simulink library "Centralized_I_Lib_Controller"  (R2024b)
(part 7 of 7)

tau = ft_14({dq1,dq2,dq3,dq4,dq5,dq6,t10,t1004,t1005,t1006,t1007,t1009,t101,t1010,t1023,t1025,t1026,t1032,t1033,t1034,t1035,t1038,t1039,t1041,t1046,t105,t1053,t106,t1063,t1068,t107,t1073,t1074,t1075,t1076,t1077,t1079,t108,t1080,t1081,t1083,t1086,t1087,t1089,t109,t1090,t1092,t1097,t1098,t11,t110,t111,t1117,t1118,t112,t1122,t1123,t1127,t1128,t113,t1130,t1131,t114,t1149,t1156,t1157,t1159,t1162,t1163,t1166,t1170,t1171,t1172,t1173,t1180,t1182,t1183,t1189,t1193,t1194,t1196,t1199,t12,t1208,t1212,t1218,t1220,t123,t1230,t1231,t1234,t1235,t1239,t124,t1243,t1244,t1245,t125,t1250,t1251,t1252,t1253,t1254,t1256,t126,t1263,t127,t1274,t128,t1287,t129,t1295,t1298,t1299,t13,t130,t1300,t1301,t1308,t1309,t1313,t1319,t1320,t1323,t1325,t1326,t1327,t1329,t1332,t1333,t1334,t1339,t1343,t1349,t1352,t1354,t1358,t1361,t1365,t1366,t1369,t1371,t1373,t1376,t1378,t1383,t1386,t1387,t1388,t1392,t1393,t1394,t1398,t140,t1406,t141,t1411,t1412,t1416,t1417,t1423,t1429,t143,t1430,t1434,t1435,t1439,t1440,t1442,t1446,t1450,t1452,t1453,t1456,t1457,t1460,t1467,t1473,t1479,t1481,t1482,t1484,t1488,t1490,t1491,t1496,t1500,t1505,t1518,t1519,t1522,t1525,t1526,t1528,t1541,t1542,t1543,t1548,t1549,t1552,t1553,t1555,t1557,t1573,t1577,t1578,t1579,t1581,t1584,t1585,t1586,t1592,t1594,t1595,t1609,t1613,t1619,t1620,t163,t164,t1642,t166,t1660,t1661,t1662,t1663,t1664,t1666,t1670,t1671,t1672,t1676,t1678,t1679,t1681,t1686,t1690,t1692,t1696,t1697,t1702,t1703,t1711,t1717,t1720,t1735,t1749,t1750,t1754,t1755,t1756,t1763,t1764,t1772,t1779,t178,t1785,t1787,t18,t1803,t1804,t1806,t1815,t1816,t182,t1820,t1824,t1826,t1827,t1828,t1829,t183,t1839,t1840,t1842,t1848,t185,t1850,t1851,t186,t1860,t1865,t1866,t1868,t1869,t1874,t1876,t1877,t1878,t1879,t1883,t189,t1895,t1898,t19,t1904,t191,t1919,t1925,t1926,t1928,t193,t1930,t1933,t194,t1942,t1947,t1949,t195,t1958,t1959,t1962,t1964,t1995,t1997,t1998,t2,t20,t200,t2000,t2002,t2003,t2004,t2014,t2017,t2018,t202,t2023,t2024,t2027,t2028,t203,t2036,t2038,t2039,t204,t2053,t2054,t2056,t2067,t2068,t2069,t2072,t2074,t2078,t208,t2086,t2087,t2094,t2096,t2097,t21,t210,t2103,t211,t2111,t2112,t2115,t212,t2124,t2125,t2126,t2127,t2132,t2138,t214,t2141,t2148,t215,t2151,t2152,t2157,t216,t2161,t2168,t2171,t2178,t2179,t2185,t22,t2201,t2205,t2208,t2212,t2217,t2221,t2222,t2223,t2224,t2225,t2227,t2229,t2231,t2236,t2237,t2238,t224,t2246,t2247,t2248,t2250,t2254,t2259,t2276,t228,t2280,t2284,t2285,t2287,t2290,t2292,t2293,t230,t2308,t231,t2320,t2324,t2343,t2347,t2348,t2358,t2362,t2373,t2375,t2383,t2387,t2394,t2395,t2397,t2398,t2400,t2401,t2403,t2404,t2405,t2409,t2411,t2412,t2417,t2419,t2421,t2422,t2423,t2426,t2432,t2433,t2439,t244,t2440,t245,t2450,t2451,t2452,t2455,t2456,t2457,t246,t2464,t2467,t247,t2472,t2473,t2474,t2477,t2478,t248,t2482,t2483,t2484,t2485,t2486,t2487,t2491,t250,t2507,t2508,t251,t252,t2527,t2529,t253,t2531,t2536,t2543,t2551,t2555,t2565,t2568,t2569,t2571,t2574,t2578,t2580,t2586,t2588,t2591,t2594,t2598,t260,t2601,t2603,t2604,t2605,t2608,t2609,t261,t2610,t2611,t2612,t2614,t2615,t262,t2622,t2625,t2629,t263,t2634,t2648,t265,t2651,t2655,t2657,t2659,t2660,t2661,t2662,t2663,t267,t2672,t2679,t2692,t2694,t2695,t2700,t2703,t2705,t2726,t2727,t2730,t2732,t2733,t2734,t2738,t2739,t2741,t2743,t2752,t2753,t2756,t2760,t2764,t2767,t2769,t2772,t2785,t2792,t2794,t2795,t2796,t28,t2804,t2806,t2809,t2811,t2815,t2817,t2819,t2820,t2821,t2825,t2829,t2830,t2832,t2833,t2836,t2839,t2843,t2844,t2848,t2850,t2852,t2856,t2861,t2862,t2863,t2866,t2869,t2877,t2878,t2880,t2888,t2890,t2892,t2899,t29,t2900,t2901,t2903,t2904,t2905,t2906,t2910,t2911,t2912,t2917,t2921,t2922,t2928,t2938,t2939,t2940,t2943,t2949,t295,t2951,t2952,t2953,t2954,t2957,t296,t2960,t2964,t297,t2970,t2977,t298,t2988,t2990,t2992,t2993,t2996,t3,t3002,t3004,t3006,t3007,t3008,t3012,t3013,t3016,t3018,t3019,t3025,t3026,t303,t3030,t3033,t3037,t3039,t304,t3040,t3043,t3045,t3046,t3047,t305,t3050,t3056,t3058,t3059,t3060,t3066,t3068,t3070,t3071,t3072,t3073,t3074,t3075,t3078,t3079,t3085,t3087,t3088,t309,t3091,t3098,t3099,t3100,t3101,t3104,t3106,t311,t3110,t3111,t312,t3129,t313,t3147,t3149,t3150,t3152,t3159,t3173,t3174,t3186,t3187,t3193,t3194,t3195,t3200,t3206,t3207,t3209,t3211,t3214,t3215,t3217,t3219,t3220,t3222,t3223,t3224,t3225,t3226,t3227,t3228,t3233,t3234,t3235,t3237,t3238,t3239,t3242,t3247,t3249,t3250,t3253,t3254,t3255,t3256,t3258,t3260,t3262,t3270,t3271,t3274,t3283,t3284,t3287,t329,t3297,t330,t3307,t3308,t331,t3323,t3326,t3327,t3328,t3329,t3330,t3331,t3335,t3336,t3345,t3346,t3348,t3353,t3359,t336,t3361,t3363,t3364,t3365,t3366,t337,t3377,t3378,t3379,t338,t3384,t3386,t339,t3394,t3395,t3396,t3397,t3405,t341,t3411,t3413,t3416,t3419,t342,t3421,t3422,t3426,t3430,t3435,t3436,t3438,t3439,t3440,t3442,t3443,t3444,t3445,t3446,t3449,t3454,t346,t3463,t3467,t3470,t3471,t3472,t3474,t3475,t3476,t3477,t348,t3480,t3481,t3488,t3491,t3492,t350,t3502,t3506,t3507,t3511,t3520,t3522,t3529,t353,t3531,t3533,t3535,t3538,t354,t3542,t3543,t3552,t3553,t356,t3565,t3566,t3567,t3568,t357,t3578,t358,t3586,t3587,t3588,t3592,t3598,t3599,t360,t3600,t3602,t3603,t3604,t3608,t3609,t3610,t3612,t3613,t3614,t3617,t3621,t3626,t3627,t3628,t3629,t3630,t3633,t3640,t3641,t3646,t3652,t3655,t3656,t3658,t3663,t3667,t3668,t3671,t3675,t3676,t3677,t3679,t3680,t3689,t369,t3691,t3692,t3697,t3698,t370,t3702,t3703,t3709,t3710,t3711,t3713,t3714,t3715,t3717,t3719,t372,t3720,t3728,t3729,t3730,t3733,t3734,t3735,t3738,t3739,t374,t3740,t3745,t3747,t3750,t3751,t3752,t3754,t3755,t3756,t3764,t3766,t3767,t3770,t3775,t3776,t3777,t3780,t3794,t3807,t3808,t3809,t3812,t3813,t3814,t3820,t3824,t3826,t3829,t3831,t384,t3841,t3852,t3854,t3856,t386,t3860,t3861,t3863,t3864,t3868,t387,t3872,t3874,t3875,t3876,t3882,t3884,t3885,t3887,t3888,t3889,t389,t3892,t3894,t3896,t3897,t3899,t3900,t3901,t3902,t3903,t3904,t3906,t3909,t3912,t3913,t3916,t3918,t3919,t3920,t3922,t3923,t3932,t3946,t3950,t3953,t3956,t3967,t3968,t397,t3970,t3972,t3981,t3982,t3985,t3993,t3994,t3998,t4,t4000,t4005,t4006,t4007,t4009,t401,t4011,t4013,t4014,t4016,t4018,t4019,t402,t4026,t4029,t4033,t4034,t4035,t4036,t4037,t404,t4044,t4046,t4047,t4048,t405,t4055,t4056,t4063,t4070,t4079,t408,t4081,t4084,t4085,t4089,t4090,t4091,t4092,t4095,t4097,t4099,t4103,t4105,t4119,t4121,t4123,t4129,t413,t4132,t4134,t4137,t4138,t414,t4140,t4142,t4143,t4145,t4147,t4148,t415,t4152,t4159,t4162,t4165,t4168,t418,t4183,t4185,t4188,t4190,t4195,t4198,t4200,t4202,t4203,t4204,t4208,t421,t4211,t4212,t4217,t4218,t4219,t4222,t4223,t4225,t4226,t4230,t4231,t4232,t4233,t4238,t4243,t4244,t4245,t4247,t4248,t4249,t425,t4250,t4252,t4265,t4271,t4276,t4277,t4280,t4282,t4284,t4287,t4292,t4294,t4295,t4301,t4305,t4309,t4310,t4311,t4313,t4316,t4317,t4319,t432,t4320,t4323,t4324,t4329,t4330,t4331,t4332,t4333,t4334,t4335,t4336,t4341,t4343,t436,t4361,t437,t4370,t4371,t4374,t4377,t4379,t4384,t4385,t4389,t439,t4390,t4391,t4399,t440,t4403,t4405,t4406,t4407,t4409,t441,t4410,t4416,t4418,t4419,t4420,t4423,t4426,t4428,t4429,t443,t4430,t4435,t444,t4442,t4444,t4448,t4449,t4452,t4454,t4457,t4471,t4473,t4477,t4478,t4479,t4484,t4493,t4495,t4496,t4499,t4507,t4514,t4518,t4519,t4526,t4528,t4533,t4536,t4538,t4539,t4540,t4546,t4547,t4550,t4551,t4554,t4556,t4557,t4559,t4562,t4571,t4573,t4574,t4575,t4579,t4581,t4582,t4584,t4592,t4594,t4595,t4597,t460,t4603,t4604,t4606,t4609,t4610,t4611,t4614,t4615,t463,t4631,t4633,t4640,t4641,t4644,t4646,t4647,t4648,t4649,t4650,t4652,t4653,t4655,t4656,t4658,t4661,t4670,t4671,t4672,t4674,t4675,t4694,t4697,t4698,t4704,t4710,t4712,t4726,t4729,t4733,t4737,t4742,t4743,t4747,t475,t4751,t4754,t4756,t4757,t4759,t4770,t4773,t4775,t4778,t478,t4780,t4782,t4784,t4785,t4786,t4787,t4794,t4797,t4798,t48,t4801,t4802,t4804,t4805,t4807,t4811,t4814,t4816,t4817,t4818,t4820,t4822,t4823,t4824,t4829,t4831,t4833,t4838,t4840,t4841,t4844,t4847,t4849,t4850,t4852,t4857,t4858,t4860,t4868,t4869,t4875,t4876,t4879,t488,t4880,t4883,t4889,t4898,t49,t4903,t4914,t4917,t4918,t4919,t4920,t4921,t4925,t4930,t4932,t4934,t494,t4940,t4942,t4946,t4949,t4950,t496,t4961,t497,t4971,t4973,t4979,t498,t4980,t4983,t4984,t4987,t4988,t499,t4995,t5,t50,t500,t501,t5010,t5026,t5030,t5032,t5036,t5039,t504,t5044,t5046,t5047,t5048,t505,t5059,t5060,t5061,t5062,t5063,t5064,t5066,t5075,t5082,t5084,t5085,t5087,t509,t5094,t5095,t5099,t51,t510,t5100,t5101,t511,t5117,t512,t5120,t5131,t5136,t5143,t5144,t5145,t5146,t5147,t5148,t515,t5153,t5156,t5158,t516,t5161,t5163,t5166,t5168,t517,t5187,t5190,t5191,t5193,t5203,t5208,t5215,t5223,t5224,t5229,t523,t5235,t524,t5242,t5244,t5250,t5252,t5265,t527,t5277,t5278,t5279,t528,t529,t5290,t5291,t5292,t5293,t5295,t5296,t5298,t53,t530,t5300,t5301,t5302,t5303,t5304,t5305,t5306,t5307,t5309,t531,t5310,t5312,t5326,t5328,t5331,t5334,t5340,t5342,t5345,t5349,t535,t5355,t536,t5360,t5364,t5365,t5366,t5371,t5372,t5375,t5376,t5377,t5382,t5384,t5388,t5389,t5393,t5394,t54,t5403,t5406,t5411,t5412,t5413,t5416,t5417,t5419,t5420,t5422,t5424,t5426,t5433,t5436,t5441,t5442,t5445,t5446,t5447,t5449,t5450,t5461,t5465,t5467,t5475,t5482,t5493,t5497,t5498,t55,t5501,t5504,t5510,t5513,t5522,t5526,t5529,t5532,t5536,t5537,t5539,t5543,t5545,t5546,t5547,t5557,t556,t5561,t557,t5573,t5576,t5579,t558,t5581,t5582,t5583,t5584,t5588,t5595,t5598,t56,t560,t5601,t5602,t5603,t5608,t5609,t5612,t5617,t5619,t562,t5620,t5622,t5627,t5628,t5629,t5630,t5631,t5637,t5646,t5647,t5648,t565,t566,t5665,t5676,t5678,t5679,t5683,t5684,t569,t57,t5701,t5705,t5719,t5720,t5722,t5724,t5729,t5730,t5732,t5735,t5736,t5747,t5749,t5753,t5756,t5757,t5759,t5762,t5776,t5778,t58,t5801,t5803,t5804,t5805,t5807,t5808,t5816,t5817,t5822,t5823,t5824,t5831,t5832,t5836,t5837,t5865,t5876,t5878,t5879,t5891,t5893,t5896,t5897,t5905,t5906,t5910,t5911,t5913,t5930,t5933,t594,t5952,t5953,t5955,t5956,t5959,t596,t5962,t5963,t5964,t5965,t5966,t5967,t5969,t5971,t5974,t5975,t5976,t5987,t5989,t599,t5990,t5995,t5999,t6,t60,t600,t6000,t6009,t6010,t6017,t6025,t6026,t6029,t6033,t6038,t6042,t6043,t6044,t605,t6051,t6052,t6054,t6055,t6058,t606,t6060,t6061,t6063,t6068,t6070,t608,t609,t6091,t61,t610,t6109,t611,t6115,t6117,t6120,t6130,t6134,t6136,t6138,t6139,t6141,t6145,t6150,t6151,t6153,t6156,t6157,t6160,t6161,t6176,t6178,t6179,t6180,t6182,t6186,t6188,t6196,t62,t6201,t6216,t6235,t6237,t6257,t6258,t6262,t6263,t6265,t6268,t6269,t6270,t6272,t6296,t63,t6302,t6313,t6317,t634,t6340,t6342,t635,t6352,t6356,t6357,t6358,t6360,t6363,t6365,t6366,t6368,t637,t638,t6386,t639,t6390,t640,t6400,t6403,t6404,t6405,t6424,t6434,t6435,t6441,t6442,t6443,t6447,t6449,t647,t6475,t6481,t6487,t649,t650,t651,t652,t6523,t6526,t653,t6531,t6533,t6534,t6549,t6562,t6563,t6564,t6570,t6576,t6586,t659,t6597,t660,t6600,t6603,t661,t663,t6635,t6638,t664,t6640,t6646,t6655,t6657,t6665,t667,t6692,t6695,t670,t6712,t6719,t6722,t6725,t6726,t6727,t6732,t6736,t6740,t6741,t6757,t676,t6760,t6763,t6764,t6766,t6770,t6771,t6775,t6776,t678,t6783,t6784,t6786,t6790,t6792,t6793,t6796,t6797,t6799,t680,t6800,t6805,t6806,t6808,t6809,t681,t6813,t6817,t6821,t6824,t6826,t6829,t6834,t684,t6843,t6845,t6849,t685,t6859,t6862,t6863,t687,t6870,t6874,t688,t6880,t6885,t6889,t6897,t690,t6905,t6906,t6909,t691,t6910,t6911,t6914,t692,t6935,t6946,t6947,t6948,t6949,t6959,t696,t6960,t6966,t6977,t6978,t6979,t6981,t6982,t6983,t6987,t7,t700,t7016,t7019,t7020,t7021,t7022,t7023,t7024,t7025,t7026,t7027,t703,t7035,t7048,t7049,t7059,t7060,t7061,t7062,t7063,t7064,t7065,t7066,t7075,t7086,t7088,t7097,t7104,t7109,t7122,t7123,t7127,t7128,t7129,t7130,t7131,t7137,t7138,t7141,t7144,t7153,t7165,t7166,t7176,t7180,t7182,t7188,t7195,t7200,t7201,t7205,t7209,t7212,t7213,t7216,t7220,t7221,t7222,t7223,t7224,t7225,t7229,t7230,t7233,t7238,t7239,t7249,t7250,t7257,t7263,t7267,t7278,t728,t7282,t7283,t7286,t7290,t7297,t7298,t7299,t7301,t7302,t7303,t7304,t7306,t7307,t7309,t7311,t7313,t7315,t7316,t7323,t7327,t7329,t7334,t7335,t7346,t7348,t735,t7357,t7358,t736,t7361,t7362,t7363,t7365,t7366,t7367,t7368,t7369,t7370,t7371,t7372,t7378,t738,t7385,t7386,t7389,t7390,t7393,t7394,t7395,t7396,t7397,t7398,t7399,t740,t7400,t7401,t7402,t7403,t7405,t7407,t7408,t7409,t7411,t7412,t7413,t7414,t7415,t7416,t7417,t7419,t7420,t7422,t7423,t7424,t7425,t7427,t7428,t7429,t7430,t7433,t7434,t7435,t7438,t7439,t7440,t7441,t7442,t7443,t7445,t7446,t7447,t7449,t7450,t7453,t7455,t7457,t746,t7460,t7461,t7463,t7464,t7465,t7466,t7467,t7469,t747,t7470,t7471,t7473,t7474,t7475,t7476,t7477,t7478,t7479,t748,t7480,t7481,t7486,t7494,t7505,t7507,t7511,t7513,t7518,t7519,t7520,t7522,t7524,t7525,t7526,t7529,t7530,t7531,t7532,t7534,t7535,t7537,t7541,t7542,t7543,t7545,t7547,t7549,t7550,t7551,t7552,t7553,t7556,t7557,t7559,t756,t7562,t7564,t7571,t7572,t7575,t7578,t7579,t758,t7580,t7582,t759,t7595,t7599,t7600,t7602,t7605,t7606,t7607,t7610,t7613,t7618,t7625,t7626,t7634,t7639,t7642,t7644,t7652,t7655,t7658,t7659,t766,t7660,t7662,t7663,t7665,t7666,t7667,t7668,t7669,t7670,t7671,t7672,t7673,t7675,t7678,t7679,t768,t7680,t7681,t7682,t7683,t7684,t7686,t7687,t7688,t7689,t7690,t7691,t7693,t7695,t7696,t7698,t7702,t7703,t7704,t7706,t7707,t7709,t7710,t7711,t7712,t7713,t7714,t7715,t7716,t7719,t772,t7720,t7721,t7722,t7723,t7725,t7739,t7741,t7742,t7743,t7745,t7746,t7747,t7748,t7749,t7750,t7752,t7753,t7755,t7756,t7757,t7758,t7759,t7764,t7765,t7769,t7770,t7773,t7774,t7775,t7777,t7793,t7802,t781,t7813,t7817,t782,t7822,t7825,t7828,t7834,t7838,t7850,t7851,t7852,t7853,t7856,t7858,t7861,t7862,t7863,t7864,t7866,t7870,t7878,t7879,t7880,t7882,t7884,t7885,t7896,t7897,t7902,t7923,t7924,t7926,t7929,t793,t7934,t7938,t7942,t7946,t7949,t7950,t7951,t7953,t7954,t7955,t7957,t7958,t7961,t7965,t7966,t7972,t7973,t7974,t7975,t7978,t798,t7981,t7984,t7985,t7987,t7988,t7989,t7990,t7992,t7993,t7994,t7995,t7998,t7999,t8,t8000,t8002,t8003,t8004,t8005,t8006,t8007,t8009,t8011,t8013,t8014,t8015,t8016,t8017,t8018,t8019,t8020,t8021,t8022,t8023,t8025,t8026,t8028,t8029,t8031,t8032,t8033,t8036,t8037,t8038,t8040,t8041,t8042,t8043,t8044,t8045,t8046,t8047,t8050,t8051,t8052,t8053,t8054,t8055,t8056,t8057,t8058,t8059,t8060,t8061,t8062,t8063,t8065,t8066,t8068,t8069,t8070,t8071,t8072,t8073,t8074,t8076,t8077,t8079,t8080,t8082,t8083,t8084,t8085,t8086,t8088,t8089,t8090,t8092,t8093,t8094,t8096,t8097,t8099,t8101,t8104,t8105,t8106,t8107,t8108,t8112,t8113,t8115,t8117,t8118,t8120,t8122,t8123,t8125,t8126,t8127,t8129,t8130,t8131,t8132,t8134,t8137,t8138,t8140,t8141,t8142,t8145,t8146,t8147,t8148,t8151,t8152,t8153,t8156,t8157,t8158,t8159,t8160,t8163,t8165,t8166,t8167,t8168,t8169,t8172,t8174,t8175,t8176,t8177,t8178,t8180,t8181,t8182,t8183,t8184,t8188,t8189,t8191,t8193,t8195,t8196,t8197,t8198,t8199,t8200,t8201,t8202,t8203,t8204,t8205,t8206,t8209,t8211,t8212,t8217,t8218,t8220,t8221,t8222,t8224,t8226,t8227,t8228,t8229,t8230,t8231,t8232,t8233,t8234,t8236,t8237,t8238,t8239,t8240,t8241,t8242,t8243,t8244,t8245,t8246,t8247,t8248,t8249,t8250,t8253,t8257,t826,t828,t829,t832,t833,t834,t836,t837,t839,t84,t85,t850,t852,t86,t861,t864,t868,t87,t879,t885,t889,t890,t891,t892,t893,t894,t897,t898,t9,t90,t900,t901,t902,t904,t905,t906,t907,t911,t912,t913,t916,t917,t92,t930,t933,t934,t936,t940,t943,t945,t947,t949,t950,t951,t956,t957,t966,t969,t97,t973,t974,t98,t981,t982,t986,t99,t992,t994,t999});
end
function tau = ft_14(ct)
[dq1,dq2,dq3,dq4,dq5,dq6,t10,t1004,t1005,t1006,t1007,t1009,t101,t1010,t1023,t1025,t1026,t1032,t1033,t1034,t1035,t1038,t1039,t1041,t1046,t105,t1053,t106,t1063,t1068,t107,t1073,t1074,t1075,t1076,t1077,t1079,t108,t1080,t1081,t1083,t1086,t1087,t1089,t109,t1090,t1092,t1097,t1098,t11,t110,t111,t1117,t1118,t112,t1122,t1123,t1127,t1128,t113,t1130,t1131,t114,t1149,t1156,t1157,t1159,t1162,t1163,t1166,t1170,t1171,t1172,t1173,t1180,t1182,t1183,t1189,t1193,t1194,t1196,t1199,t12,t1208,t1212,t1218,t1220,t123,t1230,t1231,t1234,t1235,t1239,t124,t1243,t1244,t1245,t125,t1250,t1251,t1252,t1253,t1254,t1256,t126,t1263,t127,t1274,t128,t1287,t129,t1295,t1298,t1299,t13,t130,t1300,t1301,t1308,t1309,t1313,t1319,t1320,t1323,t1325,t1326,t1327,t1329,t1332,t1333,t1334,t1339,t1343,t1349,t1352,t1354,t1358,t1361,t1365,t1366,t1369,t1371,t1373,t1376,t1378,t1383,t1386,t1387,t1388,t1392,t1393,t1394,t1398,t140,t1406,t141,t1411,t1412,t1416,t1417,t1423,t1429,t143,t1430,t1434,t1435,t1439,t1440,t1442,t1446,t1450,t1452,t1453,t1456,t1457,t1460,t1467,t1473,t1479,t1481,t1482,t1484,t1488,t1490,t1491,t1496,t1500,t1505,t1518,t1519,t1522,t1525,t1526,t1528,t1541,t1542,t1543,t1548,t1549,t1552,t1553,t1555,t1557,t1573,t1577,t1578,t1579,t1581,t1584,t1585,t1586,t1592,t1594,t1595,t1609,t1613,t1619,t1620,t163,t164,t1642,t166,t1660,t1661,t1662,t1663,t1664,t1666,t1670,t1671,t1672,t1676,t1678,t1679,t1681,t1686,t1690,t1692,t1696,t1697,t1702,t1703,t1711,t1717,t1720,t1735,t1749,t1750,t1754,t1755,t1756,t1763,t1764,t1772,t1779,t178,t1785,t1787,t18,t1803,t1804,t1806,t1815,t1816,t182,t1820,t1824,t1826,t1827,t1828,t1829,t183,t1839,t1840,t1842,t1848,t185,t1850,t1851,t186,t1860,t1865,t1866,t1868,t1869,t1874,t1876,t1877,t1878,t1879,t1883,t189,t1895,t1898,t19,t1904,t191,t1919,t1925,t1926,t1928,t193,t1930,t1933,t194,t1942,t1947,t1949,t195,t1958,t1959,t1962,t1964,t1995,t1997,t1998,t2,t20,t200,t2000,t2002,t2003,t2004,t2014,t2017,t2018,t202,t2023,t2024,t2027,t2028,t203,t2036,t2038,t2039,t204,t2053,t2054,t2056,t2067,t2068,t2069,t2072,t2074,t2078,t208,t2086,t2087,t2094,t2096,t2097,t21,t210,t2103,t211,t2111,t2112,t2115,t212,t2124,t2125,t2126,t2127,t2132,t2138,t214,t2141,t2148,t215,t2151,t2152,t2157,t216,t2161,t2168,t2171,t2178,t2179,t2185,t22,t2201,t2205,t2208,t2212,t2217,t2221,t2222,t2223,t2224,t2225,t2227,t2229,t2231,t2236,t2237,t2238,t224,t2246,t2247,t2248,t2250,t2254,t2259,t2276,t228,t2280,t2284,t2285,t2287,t2290,t2292,t2293,t230,t2308,t231,t2320,t2324,t2343,t2347,t2348,t2358,t2362,t2373,t2375,t2383,t2387,t2394,t2395,t2397,t2398,t2400,t2401,t2403,t2404,t2405,t2409,t2411,t2412,t2417,t2419,t2421,t2422,t2423,t2426,t2432,t2433,t2439,t244,t2440,t245,t2450,t2451,t2452,t2455,t2456,t2457,t246,t2464,t2467,t247,t2472,t2473,t2474,t2477,t2478,t248,t2482,t2483,t2484,t2485,t2486,t2487,t2491,t250,t2507,t2508,t251,t252,t2527,t2529,t253,t2531,t2536,t2543,t2551,t2555,t2565,t2568,t2569,t2571,t2574,t2578,t2580,t2586,t2588,t2591,t2594,t2598,t260,t2601,t2603,t2604,t2605,t2608,t2609,t261,t2610,t2611,t2612,t2614,t2615,t262,t2622,t2625,t2629,t263,t2634,t2648,t265,t2651,t2655,t2657,t2659,t2660,t2661,t2662,t2663,t267,t2672,t2679,t2692,t2694,t2695,t2700,t2703,t2705,t2726,t2727,t2730,t2732,t2733,t2734,t2738,t2739,t2741,t2743,t2752,t2753,t2756,t2760,t2764,t2767,t2769,t2772,t2785,t2792,t2794,t2795,t2796,t28,t2804,t2806,t2809,t2811,t2815,t2817,t2819,t2820,t2821,t2825,t2829,t2830,t2832,t2833,t2836,t2839,t2843,t2844,t2848,t2850,t2852,t2856,t2861,t2862,t2863,t2866,t2869,t2877,t2878,t2880,t2888,t2890,t2892,t2899,t29,t2900,t2901,t2903,t2904,t2905,t2906,t2910,t2911,t2912,t2917,t2921,t2922,t2928,t2938,t2939,t2940,t2943,t2949,t295,t2951,t2952,t2953,t2954,t2957,t296,t2960,t2964,t297,t2970,t2977,t298,t2988,t2990,t2992,t2993,t2996,t3,t3002,t3004,t3006,t3007,t3008,t3012,t3013,t3016,t3018,t3019,t3025,t3026,t303,t3030,t3033,t3037,t3039,t304,t3040,t3043,t3045,t3046,t3047,t305,t3050,t3056,t3058,t3059,t3060,t3066,t3068,t3070,t3071,t3072,t3073,t3074,t3075,t3078,t3079,t3085,t3087,t3088,t309,t3091,t3098,t3099,t3100,t3101,t3104,t3106,t311,t3110,t3111,t312,t3129,t313,t3147,t3149,t3150,t3152,t3159,t3173,t3174,t3186,t3187,t3193,t3194,t3195,t3200,t3206,t3207,t3209,t3211,t3214,t3215,t3217,t3219,t3220,t3222,t3223,t3224,t3225,t3226,t3227,t3228,t3233,t3234,t3235,t3237,t3238,t3239,t3242,t3247,t3249,t3250,t3253,t3254,t3255,t3256,t3258,t3260,t3262,t3270,t3271,t3274,t3283,t3284,t3287,t329,t3297,t330,t3307,t3308,t331,t3323,t3326,t3327,t3328,t3329,t3330,t3331,t3335,t3336,t3345,t3346,t3348,t3353,t3359,t336,t3361,t3363,t3364,t3365,t3366,t337,t3377,t3378,t3379,t338,t3384,t3386,t339,t3394,t3395,t3396,t3397,t3405,t341,t3411,t3413,t3416,t3419,t342,t3421,t3422,t3426,t3430,t3435,t3436,t3438,t3439,t3440,t3442,t3443,t3444,t3445,t3446,t3449,t3454,t346,t3463,t3467,t3470,t3471,t3472,t3474,t3475,t3476,t3477,t348,t3480,t3481,t3488,t3491,t3492,t350,t3502,t3506,t3507,t3511,t3520,t3522,t3529,t353,t3531,t3533,t3535,t3538,t354,t3542,t3543,t3552,t3553,t356,t3565,t3566,t3567,t3568,t357,t3578,t358,t3586,t3587,t3588,t3592,t3598,t3599,t360,t3600,t3602,t3603,t3604,t3608,t3609,t3610,t3612,t3613,t3614,t3617,t3621,t3626,t3627,t3628,t3629,t3630,t3633,t3640,t3641,t3646,t3652,t3655,t3656,t3658,t3663,t3667,t3668,t3671,t3675,t3676,t3677,t3679,t3680,t3689,t369,t3691,t3692,t3697,t3698,t370,t3702,t3703,t3709,t3710,t3711,t3713,t3714,t3715,t3717,t3719,t372,t3720,t3728,t3729,t3730,t3733,t3734,t3735,t3738,t3739,t374,t3740,t3745,t3747,t3750,t3751,t3752,t3754,t3755,t3756,t3764,t3766,t3767,t3770,t3775,t3776,t3777,t3780,t3794,t3807,t3808,t3809,t3812,t3813,t3814,t3820,t3824,t3826,t3829,t3831,t384,t3841,t3852,t3854,t3856,t386,t3860,t3861,t3863,t3864,t3868,t387,t3872,t3874,t3875,t3876,t3882,t3884,t3885,t3887,t3888,t3889,t389,t3892,t3894,t3896,t3897,t3899,t3900,t3901,t3902,t3903,t3904,t3906,t3909,t3912,t3913,t3916,t3918,t3919,t3920,t3922,t3923,t3932,t3946,t3950,t3953,t3956,t3967,t3968,t397,t3970,t3972,t3981,t3982,t3985,t3993,t3994,t3998,t4,t4000,t4005,t4006,t4007,t4009,t401,t4011,t4013,t4014,t4016,t4018,t4019,t402,t4026,t4029,t4033,t4034,t4035,t4036,t4037,t404,t4044,t4046,t4047,t4048,t405,t4055,t4056,t4063,t4070,t4079,t408,t4081,t4084,t4085,t4089,t4090,t4091,t4092,t4095,t4097,t4099,t4103,t4105,t4119,t4121,t4123,t4129,t413,t4132,t4134,t4137,t4138,t414,t4140,t4142,t4143,t4145,t4147,t4148,t415,t4152,t4159,t4162,t4165,t4168,t418,t4183,t4185,t4188,t4190,t4195,t4198,t4200,t4202,t4203,t4204,t4208,t421,t4211,t4212,t4217,t4218,t4219,t4222,t4223,t4225,t4226,t4230,t4231,t4232,t4233,t4238,t4243,t4244,t4245,t4247,t4248,t4249,t425,t4250,t4252,t4265,t4271,t4276,t4277,t4280,t4282,t4284,t4287,t4292,t4294,t4295,t4301,t4305,t4309,t4310,t4311,t4313,t4316,t4317,t4319,t432,t4320,t4323,t4324,t4329,t4330,t4331,t4332,t4333,t4334,t4335,t4336,t4341,t4343,t436,t4361,t437,t4370,t4371,t4374,t4377,t4379,t4384,t4385,t4389,t439,t4390,t4391,t4399,t440,t4403,t4405,t4406,t4407,t4409,t441,t4410,t4416,t4418,t4419,t4420,t4423,t4426,t4428,t4429,t443,t4430,t4435,t444,t4442,t4444,t4448,t4449,t4452,t4454,t4457,t4471,t4473,t4477,t4478,t4479,t4484,t4493,t4495,t4496,t4499,t4507,t4514,t4518,t4519,t4526,t4528,t4533,t4536,t4538,t4539,t4540,t4546,t4547,t4550,t4551,t4554,t4556,t4557,t4559,t4562,t4571,t4573,t4574,t4575,t4579,t4581,t4582,t4584,t4592,t4594,t4595,t4597,t460,t4603,t4604,t4606,t4609,t4610,t4611,t4614,t4615,t463,t4631,t4633,t4640,t4641,t4644,t4646,t4647,t4648,t4649,t4650,t4652,t4653,t4655,t4656,t4658,t4661,t4670,t4671,t4672,t4674,t4675,t4694,t4697,t4698,t4704,t4710,t4712,t4726,t4729,t4733,t4737,t4742,t4743,t4747,t475,t4751,t4754,t4756,t4757,t4759,t4770,t4773,t4775,t4778,t478,t4780,t4782,t4784,t4785,t4786,t4787,t4794,t4797,t4798,t48,t4801,t4802,t4804,t4805,t4807,t4811,t4814,t4816,t4817,t4818,t4820,t4822,t4823,t4824,t4829,t4831,t4833,t4838,t4840,t4841,t4844,t4847,t4849,t4850,t4852,t4857,t4858,t4860,t4868,t4869,t4875,t4876,t4879,t488,t4880,t4883,t4889,t4898,t49,t4903,t4914,t4917,t4918,t4919,t4920,t4921,t4925,t4930,t4932,t4934,t494,t4940,t4942,t4946,t4949,t4950,t496,t4961,t497,t4971,t4973,t4979,t498,t4980,t4983,t4984,t4987,t4988,t499,t4995,t5,t50,t500,t501,t5010,t5026,t5030,t5032,t5036,t5039,t504,t5044,t5046,t5047,t5048,t505,t5059,t5060,t5061,t5062,t5063,t5064,t5066,t5075,t5082,t5084,t5085,t5087,t509,t5094,t5095,t5099,t51,t510,t5100,t5101,t511,t5117,t512,t5120,t5131,t5136,t5143,t5144,t5145,t5146,t5147,t5148,t515,t5153,t5156,t5158,t516,t5161,t5163,t5166,t5168,t517,t5187,t5190,t5191,t5193,t5203,t5208,t5215,t5223,t5224,t5229,t523,t5235,t524,t5242,t5244,t5250,t5252,t5265,t527,t5277,t5278,t5279,t528,t529,t5290,t5291,t5292,t5293,t5295,t5296,t5298,t53,t530,t5300,t5301,t5302,t5303,t5304,t5305,t5306,t5307,t5309,t531,t5310,t5312,t5326,t5328,t5331,t5334,t5340,t5342,t5345,t5349,t535,t5355,t536,t5360,t5364,t5365,t5366,t5371,t5372,t5375,t5376,t5377,t5382,t5384,t5388,t5389,t5393,t5394,t54,t5403,t5406,t5411,t5412,t5413,t5416,t5417,t5419,t5420,t5422,t5424,t5426,t5433,t5436,t5441,t5442,t5445,t5446,t5447,t5449,t5450,t5461,t5465,t5467,t5475,t5482,t5493,t5497,t5498,t55,t5501,t5504,t5510,t5513,t5522,t5526,t5529,t5532,t5536,t5537,t5539,t5543,t5545,t5546,t5547,t5557,t556,t5561,t557,t5573,t5576,t5579,t558,t5581,t5582,t5583,t5584,t5588,t5595,t5598,t56,t560,t5601,t5602,t5603,t5608,t5609,t5612,t5617,t5619,t562,t5620,t5622,t5627,t5628,t5629,t5630,t5631,t5637,t5646,t5647,t5648,t565,t566,t5665,t5676,t5678,t5679,t5683,t5684,t569,t57,t5701,t5705,t5719,t5720,t5722,t5724,t5729,t5730,t5732,t5735,t5736,t5747,t5749,t5753,t5756,t5757,t5759,t5762,t5776,t5778,t58,t5801,t5803,t5804,t5805,t5807,t5808,t5816,t5817,t5822,t5823,t5824,t5831,t5832,t5836,t5837,t5865,t5876,t5878,t5879,t5891,t5893,t5896,t5897,t5905,t5906,t5910,t5911,t5913,t5930,t5933,t594,t5952,t5953,t5955,t5956,t5959,t596,t5962,t5963,t5964,t5965,t5966,t5967,t5969,t5971,t5974,t5975,t5976,t5987,t5989,t599,t5990,t5995,t5999,t6,t60,t600,t6000,t6009,t6010,t6017,t6025,t6026,t6029,t6033,t6038,t6042,t6043,t6044,t605,t6051,t6052,t6054,t6055,t6058,t606,t6060,t6061,t6063,t6068,t6070,t608,t609,t6091,t61,t610,t6109,t611,t6115,t6117,t6120,t6130,t6134,t6136,t6138,t6139,t6141,t6145,t6150,t6151,t6153,t6156,t6157,t6160,t6161,t6176,t6178,t6179,t6180,t6182,t6186,t6188,t6196,t62,t6201,t6216,t6235,t6237,t6257,t6258,t6262,t6263,t6265,t6268,t6269,t6270,t6272,t6296,t63,t6302,t6313,t6317,t634,t6340,t6342,t635,t6352,t6356,t6357,t6358,t6360,t6363,t6365,t6366,t6368,t637,t638,t6386,t639,t6390,t640,t6400,t6403,t6404,t6405,t6424,t6434,t6435,t6441,t6442,t6443,t6447,t6449,t647,t6475,t6481,t6487,t649,t650,t651,t652,t6523,t6526,t653,t6531,t6533,t6534,t6549,t6562,t6563,t6564,t6570,t6576,t6586,t659,t6597,t660,t6600,t6603,t661,t663,t6635,t6638,t664,t6640,t6646,t6655,t6657,t6665,t667,t6692,t6695,t670,t6712,t6719,t6722,t6725,t6726,t6727,t6732,t6736,t6740,t6741,t6757,t676,t6760,t6763,t6764,t6766,t6770,t6771,t6775,t6776,t678,t6783,t6784,t6786,t6790,t6792,t6793,t6796,t6797,t6799,t680,t6800,t6805,t6806,t6808,t6809,t681,t6813,t6817,t6821,t6824,t6826,t6829,t6834,t684,t6843,t6845,t6849,t685,t6859,t6862,t6863,t687,t6870,t6874,t688,t6880,t6885,t6889,t6897,t690,t6905,t6906,t6909,t691,t6910,t6911,t6914,t692,t6935,t6946,t6947,t6948,t6949,t6959,t696,t6960,t6966,t6977,t6978,t6979,t6981,t6982,t6983,t6987,t7,t700,t7016,t7019,t7020,t7021,t7022,t7023,t7024,t7025,t7026,t7027,t703,t7035,t7048,t7049,t7059,t7060,t7061,t7062,t7063,t7064,t7065,t7066,t7075,t7086,t7088,t7097,t7104,t7109,t7122,t7123,t7127,t7128,t7129,t7130,t7131,t7137,t7138,t7141,t7144,t7153,t7165,t7166,t7176,t7180,t7182,t7188,t7195,t7200,t7201,t7205,t7209,t7212,t7213,t7216,t7220,t7221,t7222,t7223,t7224,t7225,t7229,t7230,t7233,t7238,t7239,t7249,t7250,t7257,t7263,t7267,t7278,t728,t7282,t7283,t7286,t7290,t7297,t7298,t7299,t7301,t7302,t7303,t7304,t7306,t7307,t7309,t7311,t7313,t7315,t7316,t7323,t7327,t7329,t7334,t7335,t7346,t7348,t735,t7357,t7358,t736,t7361,t7362,t7363,t7365,t7366,t7367,t7368,t7369,t7370,t7371,t7372,t7378,t738,t7385,t7386,t7389,t7390,t7393,t7394,t7395,t7396,t7397,t7398,t7399,t740,t7400,t7401,t7402,t7403,t7405,t7407,t7408,t7409,t7411,t7412,t7413,t7414,t7415,t7416,t7417,t7419,t7420,t7422,t7423,t7424,t7425,t7427,t7428,t7429,t7430,t7433,t7434,t7435,t7438,t7439,t7440,t7441,t7442,t7443,t7445,t7446,t7447,t7449,t7450,t7453,t7455,t7457,t746,t7460,t7461,t7463,t7464,t7465,t7466,t7467,t7469,t747,t7470,t7471,t7473,t7474,t7475,t7476,t7477,t7478,t7479,t748,t7480,t7481,t7486,t7494,t7505,t7507,t7511,t7513,t7518,t7519,t7520,t7522,t7524,t7525,t7526,t7529,t7530,t7531,t7532,t7534,t7535,t7537,t7541,t7542,t7543,t7545,t7547,t7549,t7550,t7551,t7552,t7553,t7556,t7557,t7559,t756,t7562,t7564,t7571,t7572,t7575,t7578,t7579,t758,t7580,t7582,t759,t7595,t7599,t7600,t7602,t7605,t7606,t7607,t7610,t7613,t7618,t7625,t7626,t7634,t7639,t7642,t7644,t7652,t7655,t7658,t7659,t766,t7660,t7662,t7663,t7665,t7666,t7667,t7668,t7669,t7670,t7671,t7672,t7673,t7675,t7678,t7679,t768,t7680,t7681,t7682,t7683,t7684,t7686,t7687,t7688,t7689,t7690,t7691,t7693,t7695,t7696,t7698,t7702,t7703,t7704,t7706,t7707,t7709,t7710,t7711,t7712,t7713,t7714,t7715,t7716,t7719,t772,t7720,t7721,t7722,t7723,t7725,t7739,t7741,t7742,t7743,t7745,t7746,t7747,t7748,t7749,t7750,t7752,t7753,t7755,t7756,t7757,t7758,t7759,t7764,t7765,t7769,t7770,t7773,t7774,t7775,t7777,t7793,t7802,t781,t7813,t7817,t782,t7822,t7825,t7828,t7834,t7838,t7850,t7851,t7852,t7853,t7856,t7858,t7861,t7862,t7863,t7864,t7866,t7870,t7878,t7879,t7880,t7882,t7884,t7885,t7896,t7897,t7902,t7923,t7924,t7926,t7929,t793,t7934,t7938,t7942,t7946,t7949,t7950,t7951,t7953,t7954,t7955,t7957,t7958,t7961,t7965,t7966,t7972,t7973,t7974,t7975,t7978,t798,t7981,t7984,t7985,t7987,t7988,t7989,t7990,t7992,t7993,t7994,t7995,t7998,t7999,t8,t8000,t8002,t8003,t8004,t8005,t8006,t8007,t8009,t8011,t8013,t8014,t8015,t8016,t8017,t8018,t8019,t8020,t8021,t8022,t8023,t8025,t8026,t8028,t8029,t8031,t8032,t8033,t8036,t8037,t8038,t8040,t8041,t8042,t8043,t8044,t8045,t8046,t8047,t8050,t8051,t8052,t8053,t8054,t8055,t8056,t8057,t8058,t8059,t8060,t8061,t8062,t8063,t8065,t8066,t8068,t8069,t8070,t8071,t8072,t8073,t8074,t8076,t8077,t8079,t8080,t8082,t8083,t8084,t8085,t8086,t8088,t8089,t8090,t8092,t8093,t8094,t8096,t8097,t8099,t8101,t8104,t8105,t8106,t8107,t8108,t8112,t8113,t8115,t8117,t8118,t8120,t8122,t8123,t8125,t8126,t8127,t8129,t8130,t8131,t8132,t8134,t8137,t8138,t8140,t8141,t8142,t8145,t8146,t8147,t8148,t8151,t8152,t8153,t8156,t8157,t8158,t8159,t8160,t8163,t8165,t8166,t8167,t8168,t8169,t8172,t8174,t8175,t8176,t8177,t8178,t8180,t8181,t8182,t8183,t8184,t8188,t8189,t8191,t8193,t8195,t8196,t8197,t8198,t8199,t8200,t8201,t8202,t8203,t8204,t8205,t8206,t8209,t8211,t8212,t8217,t8218,t8220,t8221,t8222,t8224,t8226,t8227,t8228,t8229,t8230,t8231,t8232,t8233,t8234,t8236,t8237,t8238,t8239,t8240,t8241,t8242,t8243,t8244,t8245,t8246,t8247,t8248,t8249,t8250,t8253,t8257,t826,t828,t829,t832,t833,t834,t836,t837,t839,t84,t85,t850,t852,t86,t861,t864,t868,t87,t879,t885,t889,t890,t891,t892,t893,t894,t897,t898,t9,t90,t900,t901,t902,t904,t905,t906,t907,t911,t912,t913,t916,t917,t92,t930,t933,t934,t936,t940,t943,t945,t947,t949,t950,t951,t956,t957,t966,t969,t97,t973,t974,t98,t981,t982,t986,t99,t992,t994,t999] = ct{:};
t8139 = -t8138;
t8143 = -t8142;
t8255 = t230+t336+t354+t510+t635+t653+t681+t894+t981+t986+t1026+t1127+t1131+t1208+t1239+t1358+t1435+t1692+t1702+t1717+t2056+t2227+t2247+t2284+t2293+t2398+t2417+t2432+t2467+t2531+t2622+t2730+t2738+t2809+t2856+t2880+t3012+t3019+t3075+t3193+t3237+t3297+t3397+t3422+t3440+t3617+t3640+t3676+t3728+t3729+t3820+t3864+t3902+t4035+t4134+t4148+t4152+t4188+t4301+t4335+t4407+t4409+t4477+t4478+t4499+t4547+t4824+t4849+t4949+t5064+t5084+t5229+t5290+t5291+t5342+t5403+t5420+t5447+t5630+t5759+t5776+t5823+t5965+t6000+t6017+t6272+t7327+t7329+t7471+t7478+t7524+t7542+t8029+t8058+t8061+t8146+t8196+t8198;
et7 = t128.*(3.0./5.0e+1)-t329+t558+t599+t608-t650+t759-t826+t966+t1122-t1171+t1218+t1319+t1365+t1815-t1877+t2178+t2224-t2604+t2609+t2660+t2753+t2794+t2904+t2952+t3008+t3087+t3173+t3222+t3327+t3476+t3506+t3535+t3628+t3812+t3875-t3897+t3912+t4085+t4230+t4323+t4648+t4785+t4801+t4946+t5026+t5099+t5145+t5301+t5340+t5619+t5628+t5801+t5952+t5963+t6156+t6180+t6365-t7440-t7552+t7662-t7739-t7743+t7773+t8007+t8070+t8166+t8167+(t3755.*(t6796-t6808-t6889+t6897+t6909+t12.*t690.*(t1928-t4165).*1.35e-3))./2.0+t92.*t224-t49.*t515+(t3709.*(t7610+t688.*(t6949+t6821.*(t1928-t4165)+t6741.*(t3626-t6712))+t3.*t4.*(t6813+t7165+t6760.*(t1928-t4165))))./2.0;
et8 = (t7415.*(t7238-t7278-t7385+t3755.*(t166+t298+t2276-t2308)))./2.0+(t3754.*(-t6799+t6740.*(t1387-t3956)+t6732.*(t1552-t4983)))./2.0-t22.*t55.*t63.*1.376953125e-3-t49.*t51.*t1006.*1.6875e-2;
et9 = dq4.*(-t8248+dq6.*t8038+dq2.*t8239-dq4.*(t353+t509+t634+t651+t680+t885-t897+t917+t1035+t1081+t1098+t1130+t1183-t1326+t1369+t1371+t2290+t2394+t2529+t2796+t2877+t2957+t3018+t3072+t3284+t3336+t3405+t3419+t3435+t3600+t3863+t4145+t4185+t4320-t4336+t4405+t4495+t4540+t4726+t4820+t4857+t4920+t5063+t5158+t5235+t5422+t5446+t5504+t5805+t5816+t5822+t5990+t6263)+dq5.*(et7+et8)+dq3.*(t600+t678+t703+t828+t898+t940+t973+t1004+t1159+t1243+t1287+t1327+t1352+t1361+t1388+t1430+t1460+t1481+t1543+t1578+t1686+t1697+t1842+t1933+t2004+t2024+t2036+t2132+t2168+t2409+t2507+t2580+t2594+t2655+t2657+t2785+t2901+t2949+t3002+t3150+t3209+t3217+t3345+t3426+t3471+t3492+t3566+t3567+t3598+t3610+t3885+t3894+t3932+t3953+t4037+t4137+t4200+t4212+t4282+t4324+t4385+t4533+t4536+t4631+t4644+t4650+t4674+t4778+t4780+t4782+t4852+t4869+t4921+t4930+t5032+t5036+t5101+t5143+t5163+t5191+t5295+t5296+t5298+t5413+t5442+t5461+t5475+t5482+t5529+t5573+t5595+t5622+t5679+t5778+t5906+t5959+t5971+t6010+t6051+t6179+t6188+t6270+t6357+t6366+t6405+t6443+t6449+t6640+t8056+t8060+t8163+t8165));
et10 = -1.0;
et11 = t108.*(3.0./4.0e+1)+t112.*(3.0./4.0e+1)-t204.*(3.0./4.0e+1)-t651-t907-t1035+t1369-t2236-t2700+t3066+t3072+t3405+t3419-t4005+t4140+t4145+t4442+t4814+t4820+t5046+t5063+t5100+t5235+t5422+t5441+t5805-t3755.*(t7097+t7109+t6741.*(t1387-t3956)+t6726.*(t1928-t4165))+t690.*(t6726.*(t97-t1942)-t6732.*(t97-t1942)+t4014.*(t1387-t3956)-t4014.*(t1592-t4271))+t7.*t3767-t3709.*t7698-t7221.*t7543+t7223.*t7545+t7415.*t7453-t7419.*(t7131-t7306)+t7.*t13.*t127.*5.5078125e-3+t7.*t86.*t346.*5.625e-3+t7.*t97.*t346.*(9.0./3.2e+2)+t7.*t203.*t346.*5.625e-3;
et12 = t7.*t210.*t346.*(9.0./3.2e+2)-t7.*t13.*t63.*t97.*2.75390625e-3;
et13 = t389-t440-t441+t639+t649+t829+t891+t902-t930+t947+t956+t1032+t1079+t1092-t1123+t1170+t1180+t1194+t1411+t1429+t1442+t1542+t1581+t1595+t1676+t1679+t1696+t1755+t1764-t1816+t1820+t1840+t1876+t1904+t2000+t2003+t2127-t2179+t2208-t2223+t2229+t2387+t2588+t2605+t2692+t2911+t2939+t3104+t3159+t3195+t3223+t3247+t3260+t3271+t3323+t3474+t3522+t3609+t3656+t3691+t3794+t3861+t3874+t3884+t3896+t3946+t4103+t4119+t4123+t4208+t4252+t4277+t4280+t4361+t4384+t4538-t4649+t4747+t4805+t4831+t4838+t4875+t4879+t4898+t4903+t4918+t5153+t5278+t5328+t5364+t5412+t5417+t5532+t5536+t5561+t5579+t5648+t5678+t5701+t5735+t5747+t5753+t5803+t5836+t5896+t5905+t5969+t5974+t5987+t6026+t6029+t6043+t6063+t6130+t6136+t6139+t6161+t6178+t6201+t6216+t6313+t6363+t6386+t6404+t6435+t6442+t6447+t6475+t6481+t6487+t6531+t6576+t6635+t6655+t6657+t7439-t7520+t7719-t7741+t7742+t7853-t7864+t8015+t8074+t8076+t8172+t8175+(t7419.*(t7188+t7233-t7283-t7386))./2.0;
et14 = (t1661.*(-t6799+t6740.*(t1387-t3956)+t6732.*(t1552-t4983)))./2.0-t22.*t63.*t124.*1.376953125e-3;
et15 = t128.*(3.0./5.0e+1)-t329+t558+t599+t608-t650+t759-t826+t966+t1122-t1171+t1218+t1319+t1333+t1365+t1815-t1877+t2178+t2224-t2604+t2609+t2660+t2753+t2794+t2904+t2952+t3008+t3087+t3173+t3222+t3327+t3476+t3506+t3535+t3628+t3812+t3875-t3897+t3912+t4085+t4230+t4323+t4648+t4785+t4801+t4946+t5026+t5099+t5145+t5301+t5340+t5619+t5628+t5801+t5952+t5963+t6156+t6180+t6365-t7440-t7552+t7662-t7739-t7743+t7773+t8007+t8086+t8089+t8180+t8181+(t3755.*(t6796-t6808-t6889+t6897+t6909+t12.*t690.*(t1928-t4165).*1.35e-3))./2.0+t92.*t224+(t7415.*(t7238-t7278-t7385+t3755.*(t166+t298+t2276-t2308)))./2.0+(t3754.*(-t6799+t6740.*(t1387-t3956)+t6732.*(t1552-t4983)))./2.0;
et16 = t22.*t55.*t63.*(-1.376953125e-3)-t49.*t51.*t1006.*1.6875e-2;
et17 = t18.*1.4703625+t92+t186+t524+t528+t531+t536+t594+t676+t936+t1009-t1295-t1325+t1490+t1557-t1750-t1779+t1826+t2094+t2124+t2126+t2250+t2320+t2734+t2743+t2815+t2869+t3025+t3058+t3059+t3256+t3331+t3430+t3586+t3824+t4055+t4310+t4484+t4557+t4559+t4640+t5307+t5388+t5406+t5.*t18.*(2.7e+1./5.0e+1)-t6.*t18.*(3.0./5.0e+1)+t11.*t18.*(1.17e+2./1.0e+2)+t18.*t19.*1.180036458333333e-1-t18.*t20.*1.37635-t18.*t22.*5.5078125e-3+t18.*t63.*5.5078125e-3-t9.*t107.*(1.17e+2./1.0e+2)-t9.*t108.*(9.0./5.0e+1);
et18 = t9.*t109.*(6.0./2.5e+1)+t9.*t123.*(2.7e+1./5.0e+1)-t9.*t125.*(9.0./1.0e+2)-t49.*t85.*1.37635-t49.*t110.*(3.0./1.0e+2)-t49.*t126.*(3.0./5.0e+1)-t54.*t126.*(6.0./2.5e+1)+t9.*t204.*(9.0./5.0e+1)+t110.*t111.*5.9665625e-2+t60.*t195.*(3.0./2.5e+1)-t60.*t203.*(3.0./5.0e+1)-t86.*t195.*(3.0./2.5e+1)+t18.*t356+t19.*t691-t18.*t1006.*(9.0./8.0e+2)+t18.*t1919+t18.*t2324+t18.*t3734-t3.*t4.*t9.*(9.0./1.0e+2)+t3.*t9.*t10.*(3.9e+1./1.0e+2)+t5.*t6.*t18.*(9.0./5.0e+1)+t5.*t11.*t18.*(3.9e+1./5.0e+1)-t5.*t12.*t18.*(9.0./1.0e+2);
et19 = t18.*t19.*t21.*(-5.9665625e-2)-t18.*t19.*t22.*5.5078125e-3-t18.*t20.*t21.*5.9665625e-2+t18.*t20.*t22.*1.1015625e-2-t18.*t21.*t22.*5.5078125e-3+t4.*t9.*t49.*(3.0./2.0e+2)-t10.*t18.*t56.*(3.0./2.0e+2)-t18.*t19.*t63.*2.75390625e-3-t18.*t20.*t63.*1.1015625e-2-t18.*t21.*t63.*2.75390625e-3+t12.*t18.*t92-t18.*t50.*t58.*(9.0./1.0e+2)+t18.*t19.*t92-t18.*t50.*t62.*(6.0./2.5e+1)+t18.*t56.*t62.*(3.0./5.0e+1)-t9.*t20.*t109.*(1.2e+1./2.5e+1)+t9.*t20.*t125.*(9.0./5.0e+1);
et20 = t21.*t49.*t85.*(-5.9665625e-2)-t18.*t51.*t87.*5.9665625e-2+t22.*t49.*t85.*1.1015625e-2-t49.*t63.*t85.*1.1015625e-2-t22.*t110.*t111.*1.1015625e-2-t63.*t110.*t111.*5.5078125e-3-t13.*t18.*t346.*(9.0./1.6e+2)+t18.*t19.*t524+t18.*t19.*t676+t18.*t19.*t936-t12.*t18.*t1006.*(9.0./8.0e+2)+t18.*t20.*t1006.*(9.0./4.0e+2)+t9.*t97.*t1006.*(2.7e+1./8.0e+2)+t9.*t125.*t1006.*(9.0./1.6e+2)+t49.*t85.*t1006.*(9.0./4.0e+2)+t54.*t110.*t1006.*(9.0./1.6e+2)+t9.*t210.*t1006.*(2.7e+1./8.0e+2)+t110.*t111.*t1006.*(9.0./4.0e+2);
et21 = t60.*t203.*t1006.*(9.0./4.0e+2)+t18.*t19.*t1490+t63.*t109.*t1803+t18.*t63.*t1958+t18.*t19.*t2094+t18.*t19.*t2124+t18.*t21.*t2124+t18.*t19.*t2250+t18.*t19.*t2324+t18.*t21.*t2324+t54.*t63.*t2287+t18.*t19.*t2734+t18.*t19.*t2743+t18.*t63.*t2760+t18.*t19.*t2815+t49.*t110.*t2743+t18.*t19.*t2869+t18.*t19.*t3025+t18.*t19.*t3058+t18.*t19.*t3059+t18.*t19.*t3256+t9.*t63.*t3274+t18.*t19.*t3331+t18.*t19.*t3430+t18.*t19.*t3586+t18.*t19.*t3824+t18.*t19.*t4055+t18.*t19.*t4484+t18.*t19.*t4557+t18.*t19.*t4559+t18.*t19.*t5307+t18.*t19.*t5388+t18.*t19.*t5406+t5.*t6.*t11.*t18.*(1.2e+1./2.5e+1)-t3.*t9.*t10.*t20.*(3.9e+1./5.0e+1)-t5.*t11.*t12.*t18.*(9.0./5.0e+1)-t5.*t11.*t18.*t19.*(3.9e+1./1.0e+2)-t6.*t12.*t18.*t19.*(3.0./2.5e+1);
et22 = t6.*t12.*t18.*t20.*(-3.0./2.5e+1)+t18.*t19.*t21.*t22.*1.1015625e-2+t18.*t20.*t21.*t22.*1.1015625e-2-t4.*t9.*t21.*t49.*(3.0./2.5e+1)+t10.*t18.*t21.*t56.*(3.0./2.5e+1)+t18.*t19.*t21.*t63.*5.5078125e-3-t7.*t9.*t13.*t109.*1.1015625e-2+t21.*t22.*t49.*t85.*1.1015625e-2+t18.*t22.*t51.*t87.*1.1015625e-2+t7.*t13.*t54.*t126.*1.1015625e-2-t9.*t13.*t63.*t125.*5.5078125e-3+t21.*t49.*t63.*t85.*5.5078125e-3+t18.*t51.*t63.*t87.*5.5078125e-3-t13.*t54.*t63.*t110.*5.5078125e-3;
et23 = t22.*t63.*t110.*t111.*(-5.5078125e-3)+t7.*t63.*t86.*t195.*1.1015625e-2-t6.*t7.*t18.*t346.*(9.0./8.0e+2)-t11.*t13.*t18.*t346.*(2.7e+1./8.0e+2)+t13.*t18.*t20.*t346.*(9.0./8.0e+1)-t7.*t9.*t108.*t346.*(2.7e+1./8.0e+2)+t7.*t9.*t109.*t346.*(9.0./1.6e+2)+t9.*t13.*t107.*t346.*(2.7e+1./8.0e+2)-t9.*t13.*t125.*t346.*(9.0./8.0e+2)+t13.*t49.*t85.*t346.*(9.0./8.0e+1)-t13.*t54.*t110.*t346.*(9.0./8.0e+2)-t7.*t49.*t126.*t346.*(9.0./8.0e+2)-t7.*t54.*t126.*t346.*(9.0./1.6e+2)+t7.*t9.*t204.*t346.*(2.7e+1./8.0e+2)+t7.*t60.*t195.*t346.*(9.0./4.0e+2)+t7.*t86.*t195.*t346.*(9.0./4.0e+2);
et24 = t5.*t12.*t18.*t1006.*(2.7e+1./8.0e+2)+t12.*t18.*t20.*t1006.*(9.0./4.0e+2)-t18.*t19.*t21.*t1006.*(9.0./4.0e+2)-t18.*t20.*t21.*t1006.*(9.0./4.0e+2)+t18.*t50.*t58.*t1006.*(9.0./1.6e+2)-t18.*t51.*t61.*t1006.*(9.0./8.0e+2)-t9.*t20.*t125.*t1006.*(9.0./8.0e+1)-t21.*t49.*t85.*t1006.*(9.0./4.0e+2)-t18.*t51.*t87.*t1006.*(9.0./4.0e+2)+t49.*t63.*t85.*t1009+t50.*t62.*t63.*t1866+t18.*t19.*t63.*t1959+t49.*t63.*t85.*t1959-t5.*t6.*t11.*t18.*t19.*(6.0./2.5e+1)-t6.*t7.*t12.*t18.*t63.*5.5078125e-3-t4.*t7.*t9.*t49.*t63.*5.5078125e-3+t7.*t13.*t18.*t50.*t62.*1.1015625e-2+t7.*t10.*t18.*t56.*t63.*5.5078125e-3;
et25 = t7.*t9.*t13.*t20.*t109.*2.203125e-2-t13.*t18.*t50.*t58.*t63.*5.5078125e-3+t9.*t13.*t20.*t63.*t125.*1.1015625e-2-t3.*t9.*t10.*t13.*t346.*(9.0./8.0e+2)+t5.*t6.*t7.*t18.*t346.*(2.7e+1./8.0e+2)-t6.*t7.*t12.*t18.*t346.*(9.0./8.0e+2)-t5.*t11.*t13.*t18.*t346.*(9.0./4.0e+2)+t6.*t7.*t18.*t20.*t346.*(9.0./4.0e+2)-t4.*t7.*t9.*t49.*t346.*(9.0./8.0e+2)+t7.*t10.*t18.*t56.*t346.*(9.0./8.0e+2)-t7.*t18.*t50.*t62.*t346.*(9.0./1.6e+2)-t13.*t18.*t50.*t58.*t346.*(9.0./8.0e+2)+t7.*t18.*t56.*t62.*t346.*(9.0./8.0e+2)-t7.*t9.*t20.*t109.*t346.*(9.0./8.0e+1);
et26 = t9.*t13.*t20.*t125.*t346.*(9.0./4.0e+2)+t5.*t11.*t12.*t18.*t1006.*(9.0./8.0e+1)+t18.*t51.*t63.*t87.*t1009-t5.*t6.*t7.*t11.*t13.*t18.*2.203125e-2-t5.*t11.*t12.*t13.*t18.*t63.*1.1015625e-2+t6.*t7.*t12.*t18.*t19.*t63.*1.1015625e-2+t6.*t7.*t12.*t18.*t20.*t63.*1.1015625e-2+t4.*t7.*t9.*t21.*t49.*t63.*1.1015625e-2-t7.*t10.*t18.*t21.*t56.*t63.*1.1015625e-2+t5.*t6.*t7.*t11.*t18.*t346.*(9.0./8.0e+1)+t3.*t9.*t10.*t13.*t20.*t346.*(9.0./4.0e+2)-t5.*t11.*t12.*t13.*t18.*t346.*(9.0./4.0e+2)+t6.*t7.*t12.*t18.*t19.*t346.*(9.0./4.0e+2)+t6.*t7.*t12.*t18.*t20.*t346.*(9.0./4.0e+2);
et27 = t4.*t7.*t9.*t21.*t49.*t346.*(9.0./4.0e+2)-t7.*t10.*t18.*t21.*t56.*t346.*(9.0./4.0e+2)-t5.*t11.*t12.*t18.*t19.*t1006.*(9.0./1.6e+2)-t5.*t6.*t7.*t11.*t13.*t18.*t63.*1.1015625e-2-t5.*t6.*t7.*t11.*t18.*t19.*t346.*(9.0./1.6e+2)+2.676407291666667e-1;
et28 = t8242+dq3.*(t313+t339+t386+t885+t897+t907+t917+t934+t1035+t1081+t1128+t1183+t1263+t1326+t1371+t1386+t1412+t1456+t1577+t1672+t1749+t1898+t2426+t2464+t2752+t2796+t2957+t3046+t3066+t3258+t3284+t3336+t3405+t3600+t3711+t3770+t3981+t4018+t4079+t4081+t4105+t4140+t4320+t4336+t4442+t4457+t4540+t4704+t4726+t4814+t4857+t4876+t4920+t4934+t5046+t5082+t5100+t5158+t5235+t5372+t5422+t5441+t5647+t5736+t5805+t5831+t5837+t5990+t6033+t6134+t6263+t6296+t6600)+dq6.*t8126+dq2.*t8237-dq5.*(t250+t260+t497+t758+t837+t901+t1010+t1089+t1117+t1230+t1234+t1393+t1439+t1491+t1518+t1548+t1555+t1584+t1756+t1785+t1827+t1850+t2017+t2138+t2452+t2705+t2830+t2866+t2921+t3056+t3085+t3106+t3307+t3396+t3439+t3491+t3502+t3738+t3745+t3747+t3813+t3814+t3868+t3967+t3998+t4204+t4222+t4248+t4284+t4294+t4371+t4389+t4418+t4473+t4551+t4573+t4592+t4606+t4697+t4742+t4833+t4971+t4979+t4987+t4995+t5075+t5224+t5250+t5365+t5377+t5450+t5493+t5557+t5581+t5601+t5608+t5719+t5730+t5817+t5832+t5878+t5891+t5911+t5933+t6054+t6145+t6176+t6186+t6235+t6268+t6342+t6533+t6562+t7424+t7513+t7531+t7666+t7753+t7755+t7828+t7834+t8005+t8011+t8055+t8057+t8156+t8157);
et29 = dq4.*(t600+t678+t703+t828+t898+t940+t973+t1004+t1159+t1243+t1287+t1327+t1352+t1361+t1388+t1430+t1460+t1481+t1543+t1578+t1686+t1697+t1842+t1933+t2004+t2024+t2036+t2132+t2168+t2409+t2507+t2580+t2594+t2655+t2657+t2785+t2901+t2949+t3002+t3150+t3209+t3217+t3345+t3426+t3471+t3492+t3566+t3567+t3598+t3610+t3885+t3894+t3932+t3953+t4037+t4137+t4200+t4212+t4282+t4324+t4385+t4533+t4536+t4631+t4644+t4650+t4674+t4778+t4780+t4782+t4852+t4869+t4921+t4930+t5032+t5036+t5101+t5143+t5163+t5191+t5295+t5296+t5298+t5413+t5442+t5461+t5475+t5482+t5529+t5573+t5595+t5622+t5679+t5778+t5906+t5959+t5971+t6010+t6051+t6179+t6188+t6270+t6357+t6366+t6405+t6443+t6449+t6640+t8043+t8044+t8152+t8153);
et30 = t313+t339+t353+t386+t509+t634+t651+t680+t885+t897+t907+t917+t934+t1035+t1081+t1128+t1130+t1183+t1263+t1326+t1371+t1386+t1412+t1456+t1577+t1672+t1749+t1898+t2290+t2394+t2426+t2464+t2529+t2752+t2796+t2877+t2957+t3018+t3046+t3066+t3072+t3258+t3284+t3336+t3405+t3419+t3435+t3600+t3711+t3770+t3863+t3981+t4018+t4079+t4081+t4105+t4140+t4145+t4185+t4320+t4336+t4405+t4442+t4457+t4495+t4540+t4704+t4726+t4814+t4820+t4857+t4876+t4920+t4934+t5046+t5063+t5082+t5100+t5158+t5235+t5372+t5422+t5441+t5446+t5647+t5736+t5805+t5822+t5831+t5837+t5990+t6033+t6134+t6263+t6296+t6600+t19.*t60.*(3.0./2.0e+2)-t19.*t86.*(3.0./5.0e+1)+t19.*t112.*(9.0./1.0e+2)-t50.*t85.*(3.9e+1./1.0e+2)-t10.*t126.*(3.0./1.0e+2)+t19.*t127.*(6.0./2.5e+1)-t19.*t128.*(3.0./1.0e+2)-t62.*t110.*(3.0./2.5e+1)-t50.*t211.*(6.0./2.5e+1)+t50.*t215.*(9.0./1.0e+2)+t10.*t440+t9.*t2634+t9.*t2977+t126.*t3254+t9.*t6736;
et31 = t19.*t21.*t60.*(-3.0./2.5e+1)+t6.*t19.*t86.*5.9665625e-2-t10.*t20.*t110.*(3.0./5.0e+1)+t10.*t20.*t126.*(3.0./1.0e+2)+t20.*t62.*t440-t19.*t112.*t1006.*(9.0./1.6e+2)-t50.*t215.*t1006.*(9.0./1.6e+2)+t4.*t9.*t1720+t4.*t10.*t1895+t4.*t10.*t1925+t63.*t211.*t1947+t4.*t10.*t2472+t19.*t128.*t2743+t10.*t21.*t3211+t10.*t22.*t3211+t4.*t10.*t3233+t4.*t10.*t3253+t10.*t126.*t4055+t4.*t10.*t5305+t4.*t10.*t6068-t4.*t9.*t10.*t21.*5.9665625e-2-t6.*t19.*t22.*t86.*1.1015625e-2-t7.*t19.*t60.*t63.*5.5078125e-3-t7.*t13.*t19.*t127.*1.1015625e-2-t6.*t19.*t63.*t86.*5.5078125e-3;
et32 = t13.*t19.*t63.*t112.*5.5078125e-3+t7.*t62.*t63.*t110.*1.1015625e-2+t7.*t13.*t50.*t211.*1.1015625e-2+t13.*t50.*t63.*t215.*5.5078125e-3-t7.*t19.*t60.*t346.*(9.0./8.0e+2)-t7.*t19.*t86.*t346.*(9.0./8.0e+2)+t7.*t10.*t110.*t346.*(9.0./8.0e+2)+t13.*t19.*t112.*t346.*(9.0./8.0e+2)+t13.*t50.*t85.*t346.*(9.0./8.0e+2)+t7.*t19.*t127.*t346.*(9.0./1.6e+2)+t7.*t62.*t110.*t346.*(9.0./4.0e+2)-t7.*t50.*t211.*t346.*(9.0./1.6e+2)+t13.*t50.*t215.*t346.*(9.0./8.0e+2)+t6.*t19.*t86.*t1006.*(9.0./4.0e+2)+t4.*t9.*t20.*t1720+t4.*t10.*t22.*t1925+t4.*t9.*t20.*t2888+t10.*t21.*t22.*t3211;
et33 = t7.*t19.*t21.*t60.*t63.*1.1015625e-2-t6.*t19.*t22.*t63.*t86.*5.5078125e-3-t7.*t13.*t19.*t63.*t127.*5.5078125e-3-t7.*t20.*t62.*t63.*t110.*5.5078125e-3+t7.*t19.*t21.*t60.*t346.*(9.0./4.0e+2)-t7.*t10.*t20.*t110.*t346.*(9.0./8.0e+2)-t7.*t20.*t62.*t110.*t346.*(9.0./8.0e+2)-t4.*t9.*t10.*t21.*t1006.*(9.0./4.0e+2)+t4.*t10.*t21.*t63.*t1482+t4.*t9.*t20.*t21.*t1720;
et34 = -t389+t440+t441-t639-t649+t660-t829-t891-t902+t930-t1032-t1079+t1123+t1166+t1199+t1320+t1373+t1416+t1423+t1440+t1666-t1679+t1816+t1828+t1848+t2018+t2038+t2074+t2179-t2208+t2223+t2608+t2659+t2903+t2910+t2951+t2970+t3088+t3174+t3219-t3260+t3326+t3477+t3507+t3612+t3627+t3641+t3689-t3794+t3841+t3876+t3913+t4070+t4223+t4231+t4238+t4245+t4390+t4452+t4562+t4571+t4575+t4649+t4773+t4784+t4802+t4914+t4973+t4980+t5131+t5144+t5265+t5300+t5312+t5334+t5355+t5366+t5376+t5539+t5620+t5627+t5665+t5720+t5724+t5732+t5762+t5865+t5876+t5879+t5913+t5953+t5962+t5995+t6009+t6044+t6052+t6058+t6109+t6117+t6153+t6157+t6182+t6237+t6269+t6302+t6317+t6360+t6368+t6390+t6400+t6526+t6534+t6549+t6563+t6564+t6586+t6603+t6646+t6695+t7445+t7507+t7520+t7720+t7741+t7748+t7858+t7864+t8017+t8019-t9.*t58.*(9.0./2.0e+2)+t50.*t86.*(3.0./1.0e+2)+t9.*t129.*(9.0./2.0e+2)+t60.*t99.*(3.0./2.0e+2);
et35 = t56.*t203.*(3.0./2.5e+1)+t55.*t337+t12.*t19.*t54.*(3.0./2.0e+2)+t10.*t20.*t97.*(3.0./2.0e+2)+t10.*t20.*t108.*(3.0./1.0e+2)+t22.*t86.*t99.*5.5078125e-3+t6.*t12.*t19.*t54.*(3.0./2.5e+1)+t19.*t22.*t28.*t54.*5.5078125e-3+t7.*t13.*t20.*t126.*5.5078125e-3+t20.*t22.*t62.*t97.*5.5078125e-3+t19.*t21.*t54.*t1256+t62.*t63.*t97.*t1256+t3.*t4.*t10.*t20.*t21.*(3.0./1.0e+2);
et36 = et9.*et10-dq6.*(t8236+dq5.*t8021+dq4.*t8038+dq3.*t8126+dq2.*t8184+dq6.*(t2394+t2796+t2829+t2839+t3365+t3435+t3740+t3981+t4320+t4336+t4405+t4416+t4426+t4442+t4495+t4726+t5100+t5158+t5603))+dq1.*(dq6.*t8234+dq3.*t8240-dq5.*t8243-dq2.*t8249+dq4.*t8247)+t2487.*t7966-t2485.*t8130+t2484.*t8231-t2483.*t8238;
et37 = -dq5.*(t8244+dq6.*t8021-dq3.*(t250+t260+t497+t758+t837+t901+t1010+t1089+t1117+t1230+t1234+t1393+t1439+t1491+t1518+t1548+t1555+t1584+t1756+t1785+t1827+t1850+t2017+t2138+t2452+t2705+t2830+t2866+t2921+t3056+t3085+t3106+t3307+t3396+t3439+t3491+t3502+t3738+t3745+t3747+t3813+t3814+t3868+t3967+t3998+t4204+t4222+t4248+t4284+t4294+t4371+t4389+t4418+t4473+t4551+t4573+t4592+t4606+t4697+t4742+t4833+t4971+t4979+t4987+t4995+t5075+t5224+t5250+t5365+t5377+t5450+t5493+t5557+t5581+t5601+t5608+t5719+t5730+t5817+t5832+t5878+t5891+t5911+t5933+t6054+t6145+t6176+t6186+t6235+t6268+t6342+t6533+t6562+t7424+t7513+t7531+t7666+t7753+t7755+t7828+t7834+t8005+t8011-t8077-t8080+t8174+t8177)+dq5.*(et11+et12)-dq2.*(et13+et14)+dq4.*(et15+et16))-t2482.*(et17+et18+et19+et20+et21+et22+et23+et24+et25+et26+et27)-dq3.*(et28+et29)-dq2.*(t8250-dq2.*(et30+et31+et32+et33)+dq6.*t8184+dq3.*t8237+dq4.*t8239+dq5.*(et34+et35));
et38 = -t2486.*(t387+t511+t637+t890+t945+t1090+t1189+t1334+t1787+t1883+t2148+t2231+t2254+t2259+t2565+t2878+t2943+t3004+t3050+t3348+t3353+t3533+t3767+t3916+t4092+t4311+t4313+t4341+t4428+t4493+t4597+t4641+t4658+t4670+t4710+t4754+t4807+t5030+t5095+t5384+t5436+t5547+t5637+t7427-t3755.*t7476+t7415.*t7545-t7419.*t7543-t3709.*(-t6799+t6740.*(t1387-t3956)+t6732.*(t1552-t4983)));
et39 = t498+t556-t605-t606+t1073+t1118-t1149+t1166+t1170+t1199+t1320+t1329+t1349+t1366+t1394+t1423+t1440+t1453+t1519+t1549+t1642+t1666+t1735-t1816+t1824+t1828+t1848+t1851+t1876+t1995+t2018-t2179+t2201-t2223+t2237+t2412+t2605+t2608+t2659+t2703+t2833+t2836+t2903+t2951+t2970+t3088+t3174+t3219+t3223+t3308+t3326+t3475+t3477+t3507+t3627+t3633+t3641+t3667+t3689+t3841+t3896+t3913+t3968+t3972+t4000+t4063+t4070-t4142-t4143+t4223+t4231+t4238+t4265+t4329+t4390+t4420+t4423+t4452+t4471+t4514+t4562+t4571+t4575-t4649+t4652+t4773+t4784+t4802+t4914+t4973+t4980-t5048+t5131+t5144+t5252+t5265+t5300+t5304+t5312+t5334+t5355+t5360+t5366+t5376+t5539+t5620+t5627+t5665+t5720+t5724+t5732+t5762+t5865+t5876+t5879+t5913+t5953+t5962+t5995+t6009+t6044+t6052+t6058+t6109+t6117+t6153+t6157+t6182+t6237+t6269+t6302+t6317+t6360+t6368+t6390+t6400+t6526+t6534+t6549+t6563+t6564+t6586+t6603+t6646+t6695+t7439-t7556+t7719-t7746+t7747+t7878-t7880+t8016+t6.*t54.*(3.0./2.0e+2);
et40 = t9.*t516+t126.*t2222+t58.*t3713+(t7416.*(t7195+t7239-t7290-t7390))./2.0+(t1661.*(-t6862+t6821.*(t97-t1942)+t4014.*(t3626-t6712)))./2.0-t7.*t13.*t126.*5.5078125e-3+t49.*t51.*t61.*(9.0./2.0e+2)-t22.*t63.*t124.*1.376953125e-3-t7.*t98.*t346.*(9.0./3.2e+2)-t7.*t211.*t346.*(9.0./3.2e+2)-t9.*t62.*t1006.*1.6875e-2-t51.*t60.*t1006.*1.6875e-2-t55.*t62.*t1006.*5.625e-3-t7.*t9.*t58.*t346.*1.6875e-2;
et41 = t141+t143+t267+t312+t331+t684+t692+t834+t1025+t1039+t1086+t1196+t1376+t1392+t1496+t1526+t1541+t1681+t1868+t1997+t2014+t2023+t2067+t2383+t2478+t2629+t2727+t2863+t2928+t2996+t3101+t3149+t3207+t3386+t3411+t3470+t3520+t3565+t3588+t3621+t3658+t3680+t3720+t3856+t3909+t3950+t4132+t4211+t4218+t4243+t4309+t4370+t4379+t4614+t4770+t4797+t4961+t5087+t5120+t5166+t5190+t5203+t5242+t5331+t5345+t5419+t5424+t5467+t5497+t5588+t5617+t5705+t5757+t5893+t6141+t6196+t6258+t6356+t6424+t6523+t6638+(t7299.*(t108.*(3.0./1.0e+1)-t210.*(3.0./1.0e+1)-t384+t432+t488+t1068))./2.0+(t690.*t7413)./2.0+(t1252.*t7412)./2.0+(t1661.*t7663)./2.0-(t1703.*t7659)./2.0-(t3709.*t7429)./2.0+(t3755.*t7428)./2.0-(t6906.*t7304)./2.0+(t6905.*t7307)./2.0+(t6914.*t7301)./2.0;
et42 = t2.*(-t7618-t7884+t7929+t3709.*(t6829-t6885-t7144-t7153+t6821.*(t193-t2663)+t6151.*(t3626-t6712))+t1252.*(t6813+t7165+t6760.*(t1928-t4165))+t1661.*(t6949+t6821.*(t1928-t4165)+t6741.*(t3626-t6712))).*(-1.0./2.0)-(t8.*(t7625+t7634+t7924-t7926+t690.*(t6766+t6817+t7016-t7130+t6760.*(t189-t2612)+t6790.*(t1552-t4983))+t1252.*(-t6799+t7137+t6786.*(t1552-t4983))))./2.0+t8.*t7299.*(t7188+t7233-t7283-t7386).*(3.0./2.0)-(t8.*t7299.*(t7195+t7239-t7290-t7390))./2.0-t2.*t7304.*t7545.*(3.0./2.0)-t8.*t7304.*t7543.*(3.0./2.0)+(t2.*t7304.*t7553)./2.0;
et43 = (t8.*t7304.*t7551)./2.0-t2.*t7299.*t7882.*(3.0./2.0)+(t2.*t7299.*t7885)./2.0;
et44 = t231+t247+t342+t501+t512+t611+t670+t1076+t1156+t1173+t1212+t1332+t1354+t1450+t1670+t1879+t1962+t2423+t2456+t2569+t2611+t2662+t2769+t2850+t2906+t2954+t3111+t3200+t3225+t3228+t3329+t3359+t3384+t3538+t3552+t3630+t3646+t3698+t3715+t3751+t3900+t3920+t4011+t4089+t4226+t4334+t4519+t4526+t4579+t4584+t4610+t4656+t4787+t4829+t4950+t5147+t5303+t5371+t5382+t5522+t5546+t5631+t5683+t5967+t6038+t6060+t7298+t7303+t7358+t7411+t7423+t7525+t7668+t7669+t7675+t7678-t7681-t7683+t7765+t7769+t7950+t7955+t8079-t8158+t8218+(t3.*(-t7450+t3755.*(t6874+t7086+t3756.*(t3923-t6597))+t3709.*(-t6862+t7059+t3710.*(t3626-t6712))))./2.0+(t7370.*(t7195+t7239-t7290-t7390))./2.0+(t7885.*(t191.*(2.0./5.0)+t297+t413+t463+t504-t766-t850-t868+t1046+t1300+(t12.*t84)./1.0e+1-(t48.*t128)./1.0e+1))./2.0;
et45 = (t2.*t3.*(t7625+t7634+t7924-t7926+t690.*(t6766+t6817+t7016-t7130+t6760.*(t189-t2612)+t6790.*(t1552-t4983))+t1252.*(-t6799+t7137+t6786.*(t1552-t4983))))./2.0-(t8.*t9.*t8072)./2.0;
et46 = t252+t912+t1162+t1172+t1467-t1473+t1878+t2422+t2694+t2993+t3227+t3249-t3328+t3899+t3903+t4159+t4611+t4647+t4840-t5146+t5583+t7398-t7399-t7402-t7425+t7430-t7438+t7446-t7447+t7463+t7466-t7575+t7578+t7652+t7658+t7686+t7688+t7689-t7690-t7714-t7715-t7951-t8082+t8083+t8159+(t7885.*(t296+t369+t397+t404-t562+t728+t738-t768+t1301+t1500-(t12.*t101)./1.0e+1-(t12.*t106)./1.0e+1))./2.0+t21.*t3614;
et47 = (t1250.*(-t7618-t7884+t7929+t3709.*(t6829-t6885-t7144-t7153+t6821.*(t193-t2663)+t6151.*(t3626-t6712))+t1252.*(t6813+t7165+t6760.*(t1928-t4165))+t1661.*(t6949+t6821.*(t1928-t4165)+t6741.*(t3626-t6712))))./2.0+(t688.*(t7625+t7634+t7924-t7926+t690.*(t6766+t6817+t7016-t7130+t6760.*(t189-t2612)+t6790.*(t1552-t4983))+t1252.*(-t6799+t7137+t6786.*(t1552-t4983))))./2.0+(t7362.*(t7195+t7239-t7290-t7390))./2.0+(t4.*t9.*(-t7450+t3755.*(t6874+t7086+t3756.*(t3923-t6597))+t3709.*(-t6862+t7059+t3710.*(t3626-t6712))))./2.0;
et48 = t2.*t7299.*(t7238-t7278-t7385+t3755.*(t166+t298+t2276-t2308)).*(3.0./2.0)-t12.*t22.*t58.*5.5078125e-3-t21.*t22.*t56.*2.75390625e-3-t12.*t58.*t63.*2.75390625e-3-t21.*t56.*t63.*1.376953125e-3-t7.*t62.*t346.*5.625e-3-t28.*t56.*t1006.*5.625e-3+t12.*t58.*t2324-t7.*t10.*t28.*t63.*2.75390625e-3-t7.*t10.*t28.*t346.*5.625e-3-t5.*t7.*t62.*t346.*1.6875e-2;
et49 = t4.*(-9.0./2.0e+2)+t10.*(3.9e+1./2.0e+2)+t50.*(3.0./4.0e+2)-t57.*(9.0./1.0e+2)+t58.*(3.0./2.5e+1)+t61.*(2.7e+1./1.0e+2)-t113.*(3.0./1.0e+2)-t129.*(3.0./2.5e+1)+t130.*(9.0./1.0e+2)-t311-t350-t661+t836-t911+t2096+t2292+t2555+t2614-t2890+t3030+t3074+t3078+t3421+t3449+t3511+t3603+t3719+t3775+t3854+t4026+t4147+t4406+t4449+t4554+t4672+t4759+t4822+t4883+t5375-t5.*t10.*(1.17e+2./2.0e+2)-t10.*t20.*(3.9e+1./1.0e+2)-t5.*t61.*6.88175e-1-t21.*t50.*(3.0./5.0e+1)-t20.*t58.*(6.0./2.5e+1)-t5.*t87.*(3.0./1.0e+2)+t12.*t99.*2.98328125e-2+t20.*t348+t5.*t501;
et50 = t5.*t21.*t61.*(-2.98328125e-2)-t5.*t61.*t63.*5.5078125e-3-t12.*t22.*t99.*5.5078125e-3-t5.*t12.*t130.*(3.0./5.0e+1)-t12.*t63.*t99.*2.75390625e-3+t5.*t61.*t1009-t20.*t62.*t1006.*(9.0./1.6e+2)+t58.*t63.*t1869+t5.*t61.*t1959+t5.*t61.*t2125+t5.*t61.*t2126+t13.*t62.*t2124+t5.*t61.*t2205+t12.*t99.*t2324+t5.*t61.*t2743+t5.*t87.*t2743+t5.*t61.*t2821+t5.*t61.*t4056+t7.*t13.*t20.*t58.*1.1015625e-2+t10.*t13.*t20.*t346.*(9.0./8.0e+2)-t7.*t20.*t58.*t346.*(9.0./1.6e+2)+t13.*t20.*t62.*t346.*(9.0./8.0e+2)+t5.*t7.*t130.*t346.*(9.0./8.0e+2);
et51 = t5.*t7.*t12.*t63.*t130.*5.5078125e-3+t5.*t7.*t12.*t130.*t346.*(9.0./8.0e+2);
et52 = t8183+t8246-dq6.*t8090+dq4.*(t228+t251+t262+t443+t500+t517+t659+t663+t756+t839+t900+t943+t969+t994+t1220+t1231+t1235+t1244+t1452+t1573+t1671+t1717+t2072+t2115+t2217+t2246+t2247+t2450+t2473+t2726+t2730+t2809+t2856+t2917+t3012+t3234+t3237+t3270+t3592+t3652+t3676+t3735+t3766+t3808+t3902+t4033+t4034+t4035+t4046+t4047+t4091+t4198+t4295+t4335+t4581+t4609+t4694+t4737+t4794+t4811+t4889+t4984+t5291+t5309+t5349+t5393+t5582+t5598+t5684+t5808+t5975+t6061+t6070+t6257+t7334+t7335+t7395+t7405+t7422+t7457+t7460+t7461+t7464+t7469+t7474+t7494+t7519+t7535+t7672+t7673+t7756+t7757+t8023+t8041+t8042+t8139+t8188+t8189);
et53 = dq5.*(t231+t247+t342+t501+t512+t611+t670+t1076+t1156+t1173+t1212+t1332+t1354+t1450+t1670+t1879+t1962+t2423+t2456+t2569+t2611+t2662+t2769+t2850+t2906+t2954+t3111+t3200+t3225+t3228+t3329+t3359+t3384+t3538+t3552+t3630+t3646+t3698+t3715+t3751+t3900+t3920+t4011+t4089+t4226+t4334+t4519+t4526+t4579+t4584+t4610+t4656+t4787+t4829+t4950+t5147+t5303+t5371+t5382+t5522+t5546+t5631+t5683+t5967+t6038+t6060+t7297+t7302+t7358+t7411+t7423+t7525+t7668+t7669+t7675+t7678+t7679+t7680+t7765+t7769+t7950+t7955+t7994+t8000+t8026+t8045+t8047+t8143+t8191+t8193)-dq3.*(et49+et50+et51);
et54 = t8233+dq4.*(t50.*(9.0./4.0e+2)+t61.*(9.0./5.0e+1)-t437+t661+t836+t2358+t2756+t2804+t2844+t3449-t3511+t3675+t4009+t4090-t4147+t4332+t4430+t4449-t4554+t4672-t4883-t5.*t10.*(9.0./4.0e+1)-t12.*t99.*2.05078125e-2+t129.*t2222-t688.*t7557+t1250.*t7564-t7062.*t7064-t7063.*t7307-t2.*t7062.*(t296+t369+t397+t404-t562+t728+t738-t768+t1301+t1500-(t12.*t101)./1.0e+1-(t12.*t106)./1.0e+1).*3.0-t7.*t13.*t129.*5.5078125e-3-t12.*t99.*t1006.*(9.0./8.0e+2)+t3.*t4.*t7417+t8.*t7062.*t7362.*3.0+t2.*t7299.*t7365.*3.0+t8.*t7299.*t7367.*3.0)+dq6.*t7897;
et55 = -dq2.*(t8131+(t688.*t7429)./2.0-(t1250.*t7428)./2.0-(t7062.*t7301)./2.0-(t7061.*t7307)./2.0-t2.*t7304.*(t296+t369+t397+t404-t562+t728+t738-t768+t1301+t1500-(t12.*t101)./1.0e+1-(t12.*t106)./1.0e+1).*(3.0./2.0)+(t3.*t4.*t7413)./2.0-(t4.*t9.*t7412)./2.0+(t3.*t48.*t7663)./2.0-(t3.*t53.*t7659)./2.0+t2.*t7209.*t7299.*(3.0./2.0)+t8.*t7205.*t7299.*(3.0./2.0)+t8.*t7304.*t7362.*(3.0./2.0));
et56 = -dq3.*(t228+t251+t262+t443+t500+t517+t659+t663+t756+t839+t900+t943+t969+t994+t1220+t1231+t1235+t1244+t1452+t1573+t1671+t1717+t2072+t2115+t2217+t2246+t2247+t2450+t2473+t2726+t2730+t2809+t2856+t2917+t3012+t3234+t3237+t3270+t3592+t3652+t3676+t3735+t3766+t3808+t3902+t4033+t4034+t4035+t4046+t4047+t4091+t4198+t4295+t4335+t4581+t4609+t4694+t4737+t4794+t4811+t4889+t4984+t5291+t5309+t5349+t5393+t5582+t5598+t5684+t5808+t5975+t6061+t6070+t6257-t7327-t7329+t7395+t7405+t7422+t7457+t7460+t7461+t7464+t7470+t7475+t7494+t7518+t7534+t7672+t7673+t7756+t7757+t8028+t8059+t8145+t8195+t8197+(t8.*t9.*(t7610+t688.*(t6949+t6821.*(t1928-t4165)+t6741.*(t3626-t6712))+t3.*t4.*(t6813+t7165+t6760.*(t1928-t4165))))./2.0);
et57 = dq5.*(-t252-t912+t1406+t1417+t1473+t1711+t2039+t2225+t2661+t2953+t3224+t3328+t3443+t3614+t3629+t4202+t4247+t4249+t4448+t4615+t4786+t5047+t5059+t5146+t5302+t5629+t5966+t7393-t7394+t7402+t7425+t7433+t7438+t7447+t7449+t7465+t7467+t7575+t7579+t7655+t7660+t7687+t7690+t7691+t7693+t7706+t7707+t7949+t7951+t7989+t7992+t8032+t8063+t8147+t8200-t8203+(t1703.*(t7610+t688.*(t6949+t6821.*(t1928-t4165)+t6741.*(t3626-t6712))+t3.*t4.*(t6813+t7165+t6760.*(t1928-t4165))))./2.0+t12.*t22.*t58.*5.5078125e-3+t12.*t58.*t63.*2.75390625e-3+t58.*t63.*t1488+t7.*t10.*t28.*t63.*2.75390625e-3+t7.*t10.*t21.*t1557);
et58 = t5.*(2.7e+1./5.0e+1)+t11.*(1.17e+2./1.0e+2)-t19.*1.180036458333333e-1+t92+t186-t331+t360+t529+t1256+t1959+t2087+t2125+t2324+t2362+t2411+t2743+t2815+t2821+t3256+t3364+t4056+t5.*t6.*(9.0./5.0e+1)-t6.*t19.*(3.0./5.0e+1)-t19.*t20.*6.88175e-1+t19.*t21.*5.9665625e-2+t10.*t56.*(3.0./2.0e+2)+t50.*t58.*(9.0./1.0e+2)+t50.*t62.*(6.0./2.5e+1)-t51.*t61.*(3.0./1.0e+2)-t56.*t62.*(3.0./5.0e+1)+t51.*t87.*5.9665625e-2+t19.*t357+t19.*t436+t20.*t692;
et59 = t19.*t1006.*(-9.0./8.0e+2)+t19.*t1009+t19.*t1323+t19.*t1958+t19.*t2126+t19.*t2760+t19.*t2819+t19.*t2820+t19.*t3186+t19.*t3531+t19.*t3733+t19.*t3985+t19.*t4097+t19.*t4099+t19.*t4190+t19.*t4847+t19.*t4942+t5.*t11.*t19.*(3.9e+1./1.0e+2)+t6.*t12.*t19.*(3.0./2.5e+1)-t19.*t20.*t21.*2.98328125e-2-t19.*t21.*t22.*1.1015625e-2-t10.*t21.*t56.*(3.0./2.5e+1)-t19.*t20.*t63.*5.5078125e-3-t19.*t21.*t63.*5.5078125e-3-t22.*t51.*t87.*1.1015625e-2-t51.*t63.*t87.*5.5078125e-3-t11.*t13.*t346.*(2.7e+1./8.0e+2)+t12.*t19.*t524;
et60 = t5.*t12.*t1006.*(2.7e+1./8.0e+2)-t12.*t19.*t1006.*(9.0./8.0e+2)+t19.*t21.*t1006.*(9.0./4.0e+2)-t50.*t58.*t1006.*(9.0./1.6e+2)+t51.*t87.*t1006.*(9.0./4.0e+2)+t50.*t63.*t2111+t51.*t61.*t2743+t12.*t13.*t3206+t19.*t21.*t4055-t5.*t11.*t12.*t19.*(9.0./1.0e+2)-t19.*t21.*t22.*t63.*5.5078125e-3-t7.*t13.*t50.*t62.*1.1015625e-2-t7.*t10.*t56.*t63.*5.5078125e-3+t13.*t50.*t58.*t63.*5.5078125e-3-t22.*t51.*t63.*t87.*5.5078125e-3+t5.*t6.*t7.*t346.*(2.7e+1./8.0e+2)-t6.*t7.*t19.*t346.*(9.0./8.0e+2)-t7.*t10.*t56.*t346.*(9.0./8.0e+2);
et61 = t7.*t50.*t62.*t346.*(9.0./1.6e+2)+t13.*t50.*t58.*t346.*(9.0./8.0e+2)-t7.*t56.*t62.*t346.*(9.0./8.0e+2)+t5.*t19.*t63.*t2097-t6.*t7.*t12.*t19.*t63.*1.1015625e-2+t7.*t10.*t21.*t56.*t63.*1.1015625e-2-t6.*t7.*t12.*t19.*t346.*(9.0./4.0e+2)-t5.*t11.*t13.*t19.*t346.*(9.0./8.0e+2)+t7.*t10.*t21.*t56.*t346.*(9.0./4.0e+2)-t5.*t6.*t7.*t11.*t13.*t19.*1.1015625e-2-t5.*t11.*t12.*t13.*t19.*t346.*(9.0./8.0e+2)+1.840006875;
et62 = t498+t556-t605-t606+t1073+t1118-t1149+t1166+t1170+t1199+t1320+t1329+t1349+t1366+t1394+t1423+t1440+t1453+t1519+t1549+t1642+t1666+t1735-t1816+t1824+t1828+t1848+t1851+t1876+t1995+t2018-t2179+t2201-t2223+t2237+t2412+t2605+t2608+t2659+t2703+t2833+t2836+t2903+t2951+t2970+t3088+t3174+t3219+t3223+t3308+t3326+t3475+t3477+t3507+t3627+t3633+t3641+t3667+t3689+t3841+t3896+t3913+t3968+t3972+t4000+t4063+t4070-t4142-t4143+t4223+t4231+t4238+t4265+t4329+t4390+t4420+t4423+t4452+t4471+t4514+t4562+t4571+t4575-t4649+t4652+t4773+t4784+t4802+t4914+t4973+t4980-t5048+t5131+t5144+t5252+t5265+t5300+t5304+t5312+t5334+t5355+t5360+t5366+t5376+t5539+t5620+t5627+t5665+t5720+t5724+t5732+t5762+t5865+t5876+t5879+t5913+t5953+t5962+t5995+t6009+t6044+t6052+t6058+t6109+t6117+t6153+t6157+t6182+t6237+t6269+t6302+t6317+t6360+t6368+t6390+t6400+t6526+t6534+t6549+t6563+t6564+t6586+t6603+t6646+t6695+t7439-t7520+t7719-t7741+t7742+t7853-t7864+t8015+t6.*t54.*(3.0./2.0e+2);
et63 = t9.*t516+t126.*t2222+t58.*t3713+(t7419.*(t7188+t7233-t7283-t7386))./2.0+(t1661.*(-t6799+t6740.*(t1387-t3956)+t6732.*(t1552-t4983)))./2.0-t7.*t13.*t126.*5.5078125e-3+t49.*t51.*t61.*(9.0./2.0e+2)-t22.*t63.*t124.*1.376953125e-3-t7.*t98.*t346.*(9.0./3.2e+2)-t7.*t211.*t346.*(9.0./3.2e+2)-t9.*t62.*t1006.*1.6875e-2-t51.*t60.*t1006.*1.6875e-2-t55.*t62.*t1006.*5.625e-3-t7.*t9.*t58.*t346.*1.6875e-2;
et64 = t3.*2.8081125e+1+t49.*8.829+t54.*1.91295e+1+t85.*8.829-t110.*1.4715-t124.*1.91295e+1-t126.*2.943+t1522.*2.943-t1553.*1.4715;
et65 = -dq5.*(dq6.*t7764+dq2.*(et41+et42+et43)+dq4.*(et46+et47+et48)-dq5.*(t62.*(3.0./4.0e+1)+t311+t437+t560+t661+t2096+t2292+t2614+t3030+t3074+t3078+t3421+t3603+t3719+t3775+t3854+t4147+t4406+t4449+t4554+t4672+t4759+t4822+t690.*t7420+t3709.*t7600+t3755.*t7602-t6906.*t6914-t6910.*t7307+t2.*t6914.*t7545.*3.0+t8.*t6914.*t7543.*3.0-t2.*t7299.*t7453.*3.0-t8.*t7299.*(t7131-t7306).*3.0)+dq1.*(et39+et40)+dq3.*(et44+et45))-t4.*t9.*1.4715+t1006.*t3026.*5.518125e-1+t2487.*t7725+t2484.*t8129-t2482.*t8238;
et66 = -t2486.*(t244+t341+t496+t609+t1157+t1163+t1860+t2111+t2212+t2400+t2440+t2964+t3043+t3098+t3099+t3442+t3679+t3703+t3852+t3887+t3906+t3994+t4195+t4292+t4507+t4603+t4868+t5066-t690.*t7412+t3709.*t7663+t3755.*t7659+t6914.*t7307+t2.*t7299.*t7545.*3.0+t8.*t7299.*t7543.*3.0)-dq2.*(dq6.*t8096+dq4.*t8131+dq3.*t8182+dq5.*(t141+t143+t267+t312+t331+t684+t692+t834+t1025+t1039+t1086+t1196+t1376+t1392+t1496+t1526+t1541+t1681+t1868+t1997+t2014+t2023+t2067+t2383+t2478+t2629+t2727+t2863+t2928+t2996+t3101+t3149+t3207+t3386+t3411+t3470+t3520+t3565+t3588+t3621+t3658+t3680+t3720+t3856+t3909+t3950+t4132+t4211+t4218+t4243+t4309+t4370+t4379+t4614+t4770+t4797+t4961+t5087+t5120+t5166+t5190+t5203+t5242+t5331+t5345+t5419+t5424+t5467+t5497+t5588+t5617+t5705+t5757+t5893+t6141+t6196+t6258+t6356+t6424+t6523+t6638))-dq3.*(et52+et53)+dq4.*(et54+et55+et56+et57);
et67 = t2485.*(t10.*4.88984375e-1-t56.*(9.0./4.0e+2)+t61.*(9.0./4.0e+1)-t99.*(3.0./4.0e+1)+t248+t261+t610+t950+t1720+t2280+t2439+t2474+t2568+t2739+t2767+t2806+t2825+t2888+t3071+t3254+t3363+t3394+t3529+t3702+t3714+t3777+t3918+t3993+t4331+t4343+t4410+t4550+t4582+t4604+t4661+t4823+t4940+t5306+t5433-t10.*t21.*2.05078125e-2+t12.*t114.*2.05078125e-2+t688.*t7663+t1250.*t7659+t7062.*t7307-t2.*t7299.*(t296+t369+t397+t404-t562+t728+t738-t768+t1301+t1500-(t12.*t101)./1.0e+1-(t12.*t106)./1.0e+1).*3.0+t3.*t4.*t7412+t8.*t7299.*t7362.*3.0)-dq6.*(t8097+t8206-dq6.*(t2419+t2555+t2844+t2890+t3030+t3449+t3463+t3719+t4026+t4406+t4430+t4449+t4759)+dq5.*t7764-dq4.*t7897-dq3.*t8090)-t2483.*(et58+et59+et60+et61);
et68 = -dq1.*(-t8250+dq6.*t8202-dq4.*t8232+dq3.*t8245+dq5.*(et62+et63))-t212.*t346.*t1252.*5.518125e-1+t216.*t346.*(t126-t1522).*5.518125e-1;
et69 = t8183+t8246+dq5.*(t164+t178+t330+t350+t516+t640+t652+t832+t905+t911+t949+t974+t1038+t1087+t1173+t1434+t1457+t1690+t1879+t2423+t2508+t2591+t2695+t2912+t2940+t3228+t3250+t3287+t3346+t3602+t3613+t3692+t3826+t3900+t4129+t4138+t4546+t4841+t4925+t4932+t5117+t5168+t5279+t5394+t5537+t5584+t5756+t5807+t5976+t5999+t6265+t7297+t7302+t7358+t7411+t7423+t7525+t7668+t7669+t7675+t7678+t7679+t7680+t7765+t7769+t7950+t7955+t7994+t8000+t8026+t8045+t8047+t8143+t8191+t8193);
et70 = dq4.*(t50.*(-9.0./2.0e+2)-t56.*(9.0./5.0e+1)+t113.*(9.0./2.0e+2)+t251+t265-t500+t512+t611+t663-t839+t981+t986+t992+t1026+t1127+t1208+t1239+t1244+t1358+t1435+t1692+t1717+t2056+t2227+t2247+t2284+t2293+t2398+t2432+t2467+t2531+t2622+t2730+t2738+t2809+t2856+t2880+t3012+t3075+t3193+t3237+t3297+t3397+t3422+t3440+t3617+t3640+t3676+t3728+t3729+t3820+t3864+t3902+t4035+t4134+t4148+t4152+t4188+t4301+t4335+t4407+t4409+t4477+t4478+t4499+t4547+t4824+t4849+t4949+t5064+t5084+t5229+t5290+t5291+t5342+t5403+t5420+t5447+t5630+t5759+t5776+t5823+t5965+t6000+t6017+t6272+t7334+t7335+t7395+t7405+t7422+t7457+t7460+t7461+t7464+t7469+t7474+t7494+t7519+t7535+t7672+t7673+t7756+t7757+t8023+t8041+t8042+t8139+t8188+t8189-t12.*t130.*2.51703125e-2)+dq6.*t8050;
et71 = t647+t678+t703+t893+t916+t973+t1004+t1023+t1034+t1080+t1083+t1182+t1243+t1287+t1361+t1388+t1430+t1460+t1481+t1528+t1686+t1697+t1842+t1874+t1933+t2004+t2132+t2141+t2168+t2409+t2507+t2580+t2586+t2594+t2625+t2655+t2785+t2795+t2938+t2949+t3002+t3040+t3150+t3209+t3220+t3283+t3335+t3471+t3492+t3566+t3567+t3598+t3599+t3608+t3697+t3885+t3932+t3953+t4016+t4037+t4137+t4200+t4212+t4244+t4282+t4305+t4319+t4385+t4533+t4536+t4539+t4631+t4644+t4674+t4756+t4778+t4780+t4852+t4880+t4919+t4921+t4930+t5032+t5036+t5061+t5085+t5143+t5156+t5191+t5277+t5295+t5296+t5298+t5413+t5461+t5475+t5482+t5501+t5529+t5545+t5573+t5576+t5595+t5622+t5679+t5778+t5804+t5906+t5971+t5989+t6010+t6051+t6179+t6188+t6262+t6270+t6357+t6366+t6405+t6443+t6449+t6640-t8044+t8151+(t1250.*(-t7580+t9.*(-t6799+t7137+t6786.*(t1552-t4983))+t3.*t8.*(t6947+t6849.*(t1552-t4983)+t6740.*(t3923-t6597))))./2.0+t11.*t112.*(3.0./5.0e+1);
et72 = (t688.*(t7511+t7582+t7961-t7965+t2.*t3.*(t6947+t6849.*(t1552-t4983)+t6740.*(t3923-t6597))))./2.0+t11.*t92.*t224;
et73 = t11.*(9.0./4.0e+2)+t163+t338+t1964+t2068+t2571+t2852+t2861+t3361+t3446+t3553+t3717+t4250+t7201.*(t296+t369+t397+t404-t562+t728+t738-t768+t1301+t1500-(t12.*t101)./1.0e+1-(t12.*t106)./1.0e+1)-t7365.*(t191.*(6.0./5.0)+t305+t425+t478+t505-t781-t793-t861-t879+t1308+t12.*t84.*(3.0./1.0e+1)-t48.*t128.*(3.0./1.0e+1))+t11.*t2067+t11.*t2996+t11.*t4243+t1250.*t8118+t7367.*t7372-t688.*(t7896+t9.*(t6800+t6805+t6935-t6960-t6966+t6570.*(t1552-t4983))+t2.*t3.*(t6946+t6948-t6987-t7075+t6.*t3709.*(t1552-t4983).*1.0675e-2+t6.*t3709.*(t3626-t6712)));
et74 = -t7362.*(t200.*(3.0./1.0e+1)+t208.*(6.0./5.0)-t303-t415-t747-t1313+t12.*t105.*(3.0./1.0e+1)+t9.*t748)+t3.*t4.*(t7682-t7770+t2.*t3.*(t6834-t6843+t6863+t6870-t6959+t1664.*(t3626-t6712)))-t6.*t11.*t12.*2.05078125e-2+t6.*t12.*t1484-t3.*t4528.*t7062.*(3.0./1.0e+1)-t3.*t6719.*t7063.*(3.0./1.0e+1)-t7.*t11.*t21.*t63.*5.5078125e-3-t7.*t11.*t21.*t346.*(9.0./8.0e+2);
et75 = t358+t444+t523+t535+t696+t933+t1007+t1077+t1660+t1865+t2152+t2221+t2343+t2648+t2899+t2988+t2990+t3007+t3039+t3262+t3330+t3543+t3587+t3809+t3872+t3892+t3922+t4044+t4095+t4203+t4316+t4374+t4646+t4675+t4844+t5148+t5955-(t7371.*(t296+t369+t397+t404-t562+t728+t738-t768+t1301+t1500-(t12.*t101)./1.0e+1-(t12.*t106)./1.0e+1))./2.0+(t7369.*(t304+t372+t405+t418-t566+t740+t748-t782+t1309+t1505-t12.*t101.*(3.0./1.0e+1)-t12.*t106.*(3.0./1.0e+1)))./2.0-(t1251.*(-t7580+t9.*(-t6799+t7137+t6786.*(t1552-t4983))+t3.*t8.*(t6947+t6849.*(t1552-t4983)+t6740.*(t3923-t6597))))./2.0-(t7362.*(t214.*(3.0./1.0e+1)+t374+t414+t421+t475-t569+t746-t798-t864+t1063+t1343+t1586))./2.0;
et76 = t7200.*(t191.*(6.0./5.0)+t305+t425+t478+t505-t781-t793-t861-t879+t1308+t12.*t84.*(3.0./1.0e+1)-t48.*t128.*(3.0./1.0e+1)).*(-1.0./2.0)-(t9.*t8132)./2.0-(t687.*t8040)./2.0+(t688.*t8127)./2.0+(t7363.*(t214./1.0e+1+t370+t401+t408+t460-t565+t735-t852+t1053+t1339+t1585-(t8.*t110)./1.0e+1))./2.0-(t7370.*(t200.*(3.0./1.0e+1)+t208.*(6.0./5.0)-t303-t415-t747-t1313+t12.*t105.*(3.0./1.0e+1)+t9.*t748))./2.0+(t1250.*(t7934-t7938+t9.*(t6727+t6793+t6983+t7023-t7049+t7123)))./2.0;
et77 = (t7201.*(t191.*(2.0./5.0)+t297+t413+t463+t504-t766-t850-t868+t1046+t1300+(t12.*t84)./1.0e+1-(t48.*t128)./1.0e+1))./2.0+(t7372.*(t208.*(2.0./5.0)-t295-t402-t736+t772+t1274+(t12.*t105)./1.0e+1-(t12.*t200)./1.0e+1))./2.0+(t2.*t3.*(t7607-t7613+t7942+t688.*(t6826+t6880-t7180-t7182-t7216+t6797.*(t1552-t4983))+t10.*t7505+t3.*t4.*(t6725+t6783+t6977+t7035-t7048+t7122)))./2.0+(t3.*t10.*t8022)./2.0+(t3.*t4.*t8099)./2.0-(t3.*t8.*t8212)./2.0+t3.*t6719.*t6763.*(3.0./2.0e+1)-(t3.*t6719.*t6764)./2.0e+1+t3.*t6722.*t7062.*(3.0./2.0e+1)-(t3.*t6722.*t7065)./2.0e+1;
et78 = t647+t678+t703+t893+t916+t973+t1004+t1023+t1034+t1080+t1083+t1182+t1243+t1287+t1361+t1388+t1430+t1460+t1481+t1528+t1686+t1697+t1842+t1874+t1933+t2004+t2132+t2141+t2168+t2409+t2507+t2580+t2586+t2594+t2625+t2655+t2785+t2795+t2938+t2949+t3002+t3040+t3150+t3209+t3220+t3283+t3335+t3471+t3492+t3566+t3567+t3598+t3599+t3608+t3697+t3885+t3932+t3953+t4016+t4037+t4137+t4200+t4212+t4244+t4282+t4305+t4319+t4385+t4533+t4536+t4539+t4631+t4644+t4674+t4756+t4778+t4780+t4852+t4880+t4919+t4921+t4930+t5032+t5036+t5061+t5085+t5143+t5156+t5191+t5277+t5295+t5296+t5298+t5413+t5461+t5475+t5482+t5501+t5529+t5545+t5573+t5576+t5595+t5622+t5679+t5778+t5804+t5906+t5971+t5989+t6010+t6051+t6179+t6188+t6262+t6270+t6357+t6366+t6405+t6443+t6449+t6640-t8044+t8151+(t1250.*(-t7580+t9.*(-t6799+t7137+t6786.*(t1552-t4983))+t3.*t8.*(t6947+t6849.*(t1552-t4983)+t6740.*(t3923-t6597))))./2.0+t11.*t112.*(3.0./5.0e+1);
et79 = (t688.*(t7511+t7582+t7961-t7965+t2.*t3.*(t6947+t6849.*(t1552-t4983)+t6740.*(t3923-t6597))))./2.0+t11.*t92.*t224;
et80 = t8241+dq4.*(et78+et79)-dq2.*t8245-dq6.*(t1609+t1619+t2103+t2157+t2348+t2401+t2527+t2536+t2574+t2672+t2764+t2772+t2832+t3147+t3366+t3438+t3467+t3481+t3488+t3663+t3807+t3831+t3970+t4084+t4183+t4233+t4391+t4419+t4574+t4633+t4817+t5039+t5094+t5136+t5187+t5215+t5223+t5389+t5449+t5498+t5510+t5609+t5676+t5722+t5729+t5910+t6055+t6091+t6340+t11.*t3073+t9.*t20.*t2222+t11.*t112.*t2324+t9.*t13.*t3214-t7.*t9.*t13.*t20.*5.5078125e-3+t9.*t20.*t21.*t2222-t7.*t9.*t13.*t20.*t21.*5.5078125e-3);
et81 = dq5.*(t202.*(3.0./5.0e+1)-t250-t260-t439-t497-t758+t906-t1010+t1097+t1193-t1230-t1234+t1378+t1525-t1548+t1579+t1594+t1678+t1772+t1785+t1839+t2002+t2138+t2866+t2960+t3037+t3129+t3152+t3413+t3454+t3472+t3480+t3568+t3655+t3764+t3814+t3829+t3860+t3901+t4121+t4168+t4276+t4454+t4551+t4712+t4733+t4775+t4804+t4860+t4917+t5010+t5193+t5244+t5326+t5411+t5416+t5426+t5513+t5749+t5897+t5930+t5964+t6025+t6042+t6115+t6120+t6138+t6150+t6160+t6352+t6358+t6403+t6434+t6441+t7424+t7513+t7531+t7666+t7753+t7755+t7828+t7834+t8005+t8011+t8055+t8057+t8156+t8157+t49.*t57.*(3.0./2.0e+2)+t11.*t127.*(3.0./2.5e+1)+t51.*t111.*(3.0./5.0e+1)+t49.*t943);
et82 = t664+t999+t1254+t1479+t2086+t2285+t2433+t2733+t2741+t3013+t3047+t3238+t3730+t4479+t4751+t4798+t5310+t7127+t7229+t7311-t7346+t7473+t7481+t7532+t7537+t7704-t7711+t7716+t7973+t7974+t7975+t7987+t8025+t8053+t8054-t8085-t8088+t8092+t8101+t8106+t8107+t8122+t8125+t8229+(t6763.*(t108.*(3.0./1.0e+1)-t210.*(3.0./1.0e+1)-t384+t432+t488+t1068))./2.0+(t688.*(t7626+t7825+t7946+t3709.*(t6826+t6880-t7180-t7182-t7216+t6797.*(t1552-t4983))+t2027.*(t6947+t6849.*(t1552-t4983)+t6740.*(t3923-t6597))+t4.*t49.*(-t6799+t7137+t6786.*(t1552-t4983))))./2.0+(t7543.*(t200.*(3.0./1.0e+1)+t208.*(6.0./5.0)-t303-t415-t747-t1313+t12.*t105.*(3.0./1.0e+1)+t9.*t748))./2.0;
et83 = (t3.*t10.*(-t7450+t3755.*(t6874+t7086+t3756.*(t3923-t6597))+t3709.*(-t6862+t7059+t3710.*(t3626-t6712))))./2.0+(t3.*t4.*(t7443-t7667+t3709.*(t6784+t6806-t6978+t6981+t7021+t7024)+t3755.*(t6792+t6809-t6979+t6982+t7022+t7025)+t2027.*(t6874+t7086+t3756.*(t3923-t6597))+t1662.*(-t6862+t7059+t3710.*(t3626-t6712))))./2.0;
et84 = t183+t186+t494+t527+t531+t913+t1041+t1383+t2457+t2651+t2848+t2900+t2992+t3091+t3239+t3395+t3752+t4013+t4029+t4162+t4377+t4435+t4595+t5208+t5293+t5526+t5956-(t1662.*(-t7580+t9.*(-t6799+t7137+t6786.*(t1552-t4983))+t3.*t8.*(t6947+t6849.*(t1552-t4983)+t6740.*(t3923-t6597))))./2.0+(t7543.*(t214.*(3.0./1.0e+1)+t374+t414+t421+t475-t569+t746-t798-t864+t1063+t1343+t1586))./2.0-(t7863.*(t191.*(6.0./5.0)+t305+t425+t478+t505-t781-t793-t861-t879+t1308+t12.*t84.*(3.0./1.0e+1)-t48.*t128.*(3.0./1.0e+1)))./2.0+(t690.*t8099)./2.0-(t2027.*t8040)./2.0-(t3709.*t8127)./2.0-(t7371.*t7545)./2.0+(t7369.*t7553)./2.0+(t7372.*t7850)./2.0;
et85 = t7370.*t7862.*(-1.0./2.0)-(t7551.*(t214./1.0e+1+t370+t401+t408+t460-t565+t735-t852+t1053+t1339+t1585-(t8.*t110)./1.0e+1))./2.0+(t9.*(t7443-t7667+t3709.*(t6784+t6806-t6978+t6981+t7021+t7024)+t3755.*(t6792+t6809-t6979+t6982+t7022+t7025)+t2027.*(t6874+t7086+t3756.*(t3923-t6597))+t1662.*(-t6862+t7059+t3710.*(t3626-t6712))))./2.0-(t3755.*(t7934-t7938+t9.*(t6727+t6793+t6983+t7023-t7049+t7123)))./2.0+(t7870.*(t191.*(2.0./5.0)+t297+t413+t463+t504-t766-t850-t868+t1046+t1300+(t12.*t84)./1.0e+1-(t48.*t128)./1.0e+1))./2.0;
et86 = t2.*t3.*(t7626+t7825+t7946+t3709.*(t6826+t6880-t7180-t7182-t7216+t6797.*(t1552-t4983))+t2027.*(t6947+t6849.*(t1552-t4983)+t6740.*(t3923-t6597))+t4.*t49.*(-t6799+t7137+t6786.*(t1552-t4983))).*(-1.0./2.0)-(t3.*t6722.*(t108.*(3.0./1.0e+1)-t210.*(3.0./1.0e+1)-t384+t432+t488+t1068))./2.0e+1-(t4.*t49.*t8022)./2.0+(t3.*t8.*t8224)./2.0-t3.*t6719.*t6775.*(3.0./2.0e+1)+(t3.*t6719.*t6776)./2.0e+1-t3.*t6722.*t6914.*(3.0./2.0e+1);
et87 = -dq4.*(et82+et83)-dq1.*(t202.*(3.0./5.0e+1)-t250-t260-t439-t497-t758+t906+t1033+t1097+t1193+t1298+t1378+t1525-t1548+t1579+t1594+t1678+t1772+t1785+t1839+t2002+t2138+t2866+t2960+t3037+t3129+t3152+t3413+t3454+t3472+t3480+t3568+t3655+t3764+t3814+t3829+t3860+t3901+t4121+t4168+t4276+t4454+t4551+t4712+t4733+t4775+t4804+t4860+t4917+t5010+t5193+t5244+t5326+t5411+t5416+t5426+t5513+t5749+t5897+t5930+t5964+t6025+t6042+t6115+t6120+t6138+t6150+t6160+t6352+t6358+t6403+t6434+t6441+t7424+t7550+t7562+t7666+t7758+t7759+t7852+t7856+t8006+t8013+t8055+t8057+t8156+t8157+t11.*t127.*(3.0./2.5e+1)+t51.*t111.*(3.0./5.0e+1)-t9.*t685+t49.*t943+t9.*t12.*t20.*(3.0./1.0e+2))+dq6.*t7442;
et88 = dq2.*(t164+t178+t330+t350+t516+t640+t652+t832+t905+t911+t949+t974+t1038+t1087+t1173+t1434+t1457+t1690+t1879+t2423+t2508+t2591+t2695+t2912+t2940+t3228+t3250+t3287+t3346+t3602+t3613+t3692+t3826+t3900+t4129+t4138+t4546+t4841+t4925+t4932+t5117+t5168+t5279+t5394+t5537+t5584+t5756+t5807+t5976+t5999+t6265+t7297+t7302+t7357+t7409+t7670+t7671+t7679+t7680+t7953+t7957+t7994+t8000+t8026+t8045+t8047+t8143+t8191+t8193+t8226+t8227)+dq3.*(et84+et85+et86);
et89 = dq5.*(t163+t1964+t3361+t3446+t3553+t3717+t4250-t7453.*(t191.*(6.0./5.0)+t305+t425+t478+t505-t781-t793-t861-t879+t1308+t12.*t84.*(3.0./1.0e+1)-t48.*t128.*(3.0./1.0e+1))-t6.*t11.*(3.0./2.0e+2)-t3709.*t8104+t7213.*t7545-t7225.*t7543+t690.*(t7606-t7702+t3.*t8.*(t7060-t7088+t7104+t3710.*(t3923-t6597)))+t7372.*(t7131-t7306)-t3755.*(-t7813+t9.*(t7138-t7166+t7176+t6757.*(t1928-t4165))+t3.*t8.*(t7257+t7267+t6824.*(t1928-t4165)+t6741.*(t3923-t6597)))+t90.*t4219.*t6914+t90.*t6719.*t6910+t5.*t6.*t13.*t1557+t5.*t7.*t12.*t13.*t63.*2.75390625e-3);
et90 = t109.*(-1.4715)-t125.*2.943-t194.*2.943+t202.*1.4715;
et91 = -t2485.*(t185+t246+t309+t1398+t2053+t2112+t2151+t2373+t2404+t2817+t3045+t3100+t3187+t3378+t3445+t3542+t3889+t4217+t4556+t5044-t688.*(-t7580+t9.*(-t6799+t7137+t6786.*(t1552-t4983))+t3.*t8.*(t6947+t6849.*(t1552-t4983)+t6740.*(t3923-t6597)))-t1250.*t8040+t7362.*t7372+(t296+t369+t397+t404-t562+t728+t738-t768+t1301+t1500-(t12.*t101)./1.0e+1-(t12.*t106)./1.0e+1).*(t191.*(6.0./5.0)+t305+t425+t478+t505-t781-t793-t861-t879+t1308+t12.*t84.*(3.0./1.0e+1)-t48.*t128.*(3.0./1.0e+1))-t3.*t4.*t8022+t90.*t6719.*t7062)-t3.*t10.*1.4715+t4.*t49.*1.91295e+1;
et92 = t4.*t54.*(-8.829)+t1006.*t2028.*5.518125e-1-t2487.*t7403+t2483.*t8129+t2482.*t8231+dq2.*(et69+et70);
et93 = -dq4.*(dq6.*t7526-dq3.*(et75+et76+et77)+dq5.*(t664+t999+t1254+t1479+t2086+t2285+t2433+t2733+t2741+t3013+t3047+t3238+t3730+t4479+t4751+t4798+t5310+t7127+t7229+t7311+t7316+t7348+t7473+t7481+t7532+t7537+t7972+t7973+t7974+t7985+t8025+t8031+t8053+t8054+t8066+t8068+t8092+t8101+t8106+t8107+t8122+t8125+t8134+t8217+t8220)-dq2.*(t230+t336+t354+t510+t635+t653+t681+t894+t981+t986+t1026+t1127+t1131+t1208+t1239+t1358+t1435+t1692+t1702+t1717+t2056+t2227+t2247+t2284+t2293+t2398+t2417+t2432+t2467+t2531+t2622+t2730+t2738+t2809+t2856+t2880+t3012+t3019+t3075+t3193+t3237+t3297+t3397+t3422+t3440+t3617+t3640+t3676+t3728+t3729+t3820+t3864+t3902+t4035+t4134+t4148+t4152+t4188+t4301+t4335+t4407+t4409+t4477+t4478+t4499+t4547+t4824+t4849+t4949+t5064+t5084+t5229+t5290+t5291+t5342+t5403+t5420+t5447+t5630+t5759+t5776+t5823+t5965+t6000+t6017+t6272+t7334+t7335+t7469+t7474+t7519+t7535+t8023+t8041+t8042+t8139+t8188+t8189)+dq1.*(et71+et72)+dq4.*(et73+et74));
et94 = dq3.*(dq6.*t7793+dq5.*(t183+t186+t494+t527+t531+t913+t1041+t1383+t2457+t2651+t2848+t2900+t2992+t3091+t3239+t3395+t3752+t4013+t4029+t4162+t4377+t4435+t4595+t5208+t5293+t5526+t5956)+dq4.*(t358+t444+t523+t535+t696+t933+t1007+t1077+t1660+t1865+t2152+t2221+t2343+t2648+t2899+t2988+t2990+t3007+t3039+t3262+t3330+t3543+t3587+t3809+t3872+t3892+t3922+t4044+t4095+t4203+t4316+t4374+t4646+t4675+t4844+t5148+t5955))-dq1.*(et80+et81);
et95 = t2486.*(t245+t263+t667+t1484+t1926+t1949+t2403+t2477+t2811+t3255+t3379+t3444+t3671+t3888+t3919-t3709.*(-t7580+t9.*(-t6799+t7137+t6786.*(t1552-t4983))+t3.*t8.*(t6947+t6849.*(t1552-t4983)+t6740.*(t3923-t6597)))-t7545.*(t191.*(6.0./5.0)+t305+t425+t478+t505-t781-t793-t861-t879+t1308+t12.*t84.*(3.0./1.0e+1)-t48.*t128.*(3.0./1.0e+1))+t690.*t8022-t3755.*t8040+t7372.*t7543+t90.*t6719.*t6914)+dq6.*(t7802+t8052+t8117+dq5.*t7442-dq4.*t7526+dq6.*(t2068+t2375+t2861+t3361+t3377+t3446));
et96 = -t2484.*(t92+t186+t524+t531+t536+t594+t676+t936+t1009+t1490+t1557+t2094+t2124+t2126+t2250+t2734+t2743+t2815+t2869+t3025+t3058+t3059+t3256+t3331+t3430+t3586+t3824+t4055+t4310+t4484+t4557+t4559+t4640+t5307+t5388+t5406+2.362807291666667e-1)+dq5.*(et87+et88+et89)+t216.*t346.*t1663.*5.518125e-1-t4.*t49.*t212.*t346.*5.518125e-1;
et97 = t141+t143+t267+t1868+t2023+t2067+t2478+t2727+t2863+t2996+t3588+t3621+t3856+t4243+(t7063.*(t108.*(3.0./1.0e+1)-t210.*(3.0./1.0e+1)-t384+t432+t488+t1068))./2.0+(t690.*(-t7684+t7777+t688.*(t6834-t6843+t6863+t6870-t6959+t1664.*(t3626-t6712))))./2.0-(t1253.*(t7435+t1250.*(t6874+t7086+t3756.*(t3923-t6597))+t688.*(-t6862+t7059+t3710.*(t3626-t6712))))./2.0+(t1250.*t8199)./2.0-(t3709.*t8123)./2.0-(t3755.*t8120)./2.0-(t6771.*t7062)./2.0+(t6770.*t7065)./2.0+(t6914.*t7066)./2.0-(t7366.*t7545)./2.0-(t7368.*t7543)./2.0+(t7365.*t7553)./2.0+(t7367.*t7551)./2.0+(t7363.*t7851)./2.0-(t7362.*t7866)./2.0;
et98 = t3060.*(t7610+t688.*(t6949+t6821.*(t1928-t4165)+t6741.*(t3626-t6712))+t3.*t4.*(t6813+t7165+t6760.*(t1928-t4165))).*(-1.0./2.0)-((t7249-t7282-t7389+t3755.*(t166+t298+t2276-t2308).*3.0).*(t296+t369+t397+t404-t562+t728+t738-t768+t1301+t1500-(t12.*t101)./1.0e+1-(t12.*t106)./1.0e+1))./2.0+((t7238-t7278-t7385+t3755.*(t166+t298+t2276-t2308)).*(t304+t372+t405+t418-t566+t740+t748-t782+t1309+t1505-t12.*t101.*(3.0./1.0e+1)-t12.*t106.*(3.0./1.0e+1)))./2.0;
et99 = t688.*(t7559+t7642+t7644-t7923+t3709.*(t6946+t6948-t6987-t7075+t6.*t3709.*(t1552-t4983).*1.0675e-2+t6.*t3709.*(t3626-t6712))+t690.*(t6800+t6805+t6935-t6960-t6966+t6570.*(t1552-t4983))).*(-1.0./2.0)+(t3754.*(t7522+t7605+t1250.*(t6947+t6849.*(t1552-t4983)+t6740.*(t3923-t6597))))./2.0+(t3.*t4.*t8140)./2.0;
et100 = dq2.*(t252+t261+t530+t557+t610+t700+t904+t912+t950+t1075+t1172+t1878+t2171+t2238+t2397+t2422+t2491+t2610+t2661+t2843+t2905+t2953+t3006+t3215+t3224+t3227+t3328+t3443+t3578+t3629+t3668+t3899+t4202+t4249+t4287+t4333+t4429+t4594+t4615+t4655+t4786+t5059+t5146+t5302+t5629+t5966+t7394+t7399+t7401+t7407+t7695+t7696+t7710+t7712+t7954+t7958+t7990+t7995+t8033+t8062+t8065+t8148+t8201+t8203+t8204+t8209);
et101 = dq5.*(t12.*(-3.0./4.0e+1)+t2078+t2892-t7453.*(t304+t372+t405+t418-t566+t740+t748-t782+t1309+t1505-t12.*t101.*(3.0./1.0e+1)-t12.*t106.*(3.0./1.0e+1))+t6.*t957-t12.*t1006.*(9.0./3.2e+2)+t13.*t2054-t690.*t8093+t3709.*t8108+t6771.*t6914+t6910.*t7065-t7020.*t7545+t7027.*t7543+t7363.*(t7131-t7306)+t3755.*(t7838+t1250.*(t7257+t7267+t6824.*(t1928-t4165)+t6741.*(t3923-t6597))+t3.*t4.*(t7138-t7166+t7176+t6757.*(t1928-t4165)))-t6.*t7.*t346.*(9.0./3.2e+2))-dq6.*t7323;
et102 = -dq1.*(t499+t511+t558+t599+t608+t759+t966+t1074+t1090+t1171+t1218+t1299+t1319+t1333+t1365+t1877+t1998+t2347+t2421+t2455+t2604+t2609+t2660+t2753+t2794+t2904+t2922+t2952+t3008+t3087+t3110+t3173+t3222+t3226+t3327+t3476+t3506+t3535+t3628+t3739+t3750+t3812+t3897+t3912+t4006+t4085+t4225+t4230+t4232+t4323+t4330+t4518+t4653+t4698+t4743+t4785+t4801+t4946+t4988+t5026+t5060+t5145+t5301+t5340+t5543+t5602+t5619+t5628+t5801+t5824+t5952+t5963+t6156+t6180+t6365+t7440+t7571+t7572+t7665+t7745+t7752+t7817+t7822+t8004+t8014+t8069+t8071+t8168+t8169)-dq4.*(et97+et98+et99)+dq3.*(t182+t253+t664+t1005+t1245+t1479+t2086+t2097+t2248+t2451+t2615+t2732+t2733+t2792+t3016+t3033+t3079+t3238+t3604+t3677+t3776+t3904+t4036+t4048+t4317+t4850+t5292+t7230+t7313+t7316+t7348+t7477+t7479+t7530+t7541-t7704+t7709+t7711+t7713./2.0+t7972+t7981+t7984+t7985+t8031+t8066+t8068+t8094+t8112+t8113+t8134+t8141+t8205+t8211+t8217+t8220);
et103 = t8233-dq2.*t8131+dq3.*t8255+dq6.*(t1613+t1620-t2161+t2185+t2395+t2405+t2578+t2679+t3436-t3442+t3882-t4007+t4399+t4496+t21.*t1804+t21.*t2598+t21.*t2601-t22.*t63.*t113.*1.376953125e-3-t7.*t10.*t346.*(9.0./3.2e+2)-t12.*t13.*t58.*t63.*2.75390625e-3-t12.*t13.*t58.*t346.*5.625e-3-t13.*t21.*t56.*t346.*5.625e-3);
et104 = -dq5.*(t252+t261+t530+t557+t610+t700+t904+t912+t950+t1075+t1172+t1878+t2171+t2238+t2397+t2422+t2491+t2610+t2661+t2843+t2905+t2953+t3006+t3215+t3224+t3227+t3328+t3443+t3578+t3629+t3668+t3899+t4202+t4249+t4287+t4333+t4429+t4594+t4615+t4655+t4786+t5059+t5146+t5302+t5629+t5966+t7394-t7408+t7430-t7438-t7575+t7578+t7686+t7688+t7689-t7690+t7710+t7712-t7951+t7990+t7995+t8033+t8062+t8065+t8148+t8201+t8203+t2.*t7299.*(t7238-t7278-t7385+t3755.*(t166+t298+t2276-t2308)).*(3.0./2.0));
et105 = -dq4.*(t50.*(-3.0./2.0e+2)+t61.*(9.0./2.0e+2)+t114.*(3.0./5.0e+1)+t129.*(3.0./5.0e+1)-t248+t560+t609-t661+t951+t21.*t50.*(3.0./1.0e+2)-t12.*t99.*4.6625e-3+(t688.*t7557)./2.0-(t1250.*t7564)./2.0+(t7062.*t7064)./2.0+(t7063.*t7307)./2.0+t2.*t7062.*(t296+t369+t397+t404-t562+t728+t738-t768+t1301+t1500-(t12.*t101)./1.0e+1-(t12.*t106)./1.0e+1).*(3.0./2.0)-(t3.*t4.*t7417)./2.0-t8.*t7062.*t7362.*(3.0./2.0)-t2.*t7299.*t7365.*(3.0./2.0)-t8.*t7299.*t7367.*(3.0./2.0));
et106 = t8248-dq3.*(t647+t678+t703+t828+t893+t916+t973+t1004+t1023+t1034+t1080+t1182+t1243+t1287+t1361+t1388+t1430+t1460+t1481+t1528+t1543+t1686+t1697-t1829+t1874+t1933+t2132+t2141+t2168+t2409+t2507+t2580+t2586+t2594+t2625+t2655+t2785+t2795+t2938+t2949+t3002+t3040+t3150+t3209+t3220+t3283+t3335+t3471+t3492+t3566+t3567+t3598+t3599+t3608+t3697+t3885+t3932+t3953+t4016+t4037+t4137+t4200+t4212+t4244+t4282+t4305+t4319+t4385+t4533+t4536+t4539+t4631+t4644+t4674+t4756+t4778+t4780+t4852+t4880+t4919+t4921+t4930+t5032+t5036+t5061+t5085+t5143+t5156+t5191+t5277+t5295+t5296+t5298+t5413+t5461+t5475+t5482+t5501+t5529+t5545+t5573+t5576+t5595+t5622+t5679+t5778+t5804+t5906+t5971+t5989+t6010+t6051+t6179+t6188+t6262+t6270+t6357+t6366+t6405+t6443+t6449+t6640+t8056+t8060+t8163+t8165+t12.*t600+t12.*t1446)+dq6.*t8046+dq2.*t8232;
et107 = dq5.*(t499+t511+t558+t599+t608+t759+t966+t1074+t1090+t1171+t1218+t1299+t1319+t1333+t1365+t1877+t1998+t2347+t2421+t2455+t2604+t2609+t2660+t2753+t2794+t2904+t2922+t2952+t3008+t3087+t3110+t3173+t3222+t3226+t3327+t3476+t3506+t3535+t3628+t3739+t3750+t3812+t3897+t3912+t4006+t4085+t4225+t4230+t4232+t4323+t4330+t4518+t4653+t4698+t4743+t4785+t4801+t4946+t4988+t5026+t5060+t5145+t5301+t5340+t5543+t5602+t5619+t5628+t5801+t5824+t5952+t5963+t6156+t6180+t6365+t7440+t7549+t7552+t7665+t7739+t7743+t7774+t7775+t8003+t8009+t8069+t8071+t8168+t8169);
et108 = t185+t246+t309+t1398+t2053+t2112+t2151+t2373+t2404+t2817+t3045+t3100+t3187+t3378+t3445+t3542+t3889+t4217+t4556+t5044-t9.*(t7435+t1250.*(t6874+t7086+t3756.*(t3923-t6597))+t688.*(-t6862+t7059+t3710.*(t3626-t6712)))+t7363.*t7370+(t304+t372+t405+t418-t566+t740+t748-t782+t1309+t1505-t12.*t101.*(3.0./1.0e+1)-t12.*t106.*(3.0./1.0e+1)).*(t191.*(2.0./5.0)+t297+t413+t463+t504-t766-t850-t868+t1046+t1300+(t12.*t84)./1.0e+1-(t48.*t128)./1.0e+1)+t2.*t3.*(t7522+t7605+t1250.*(t6947+t6849.*(t1552-t4983)+t6740.*(t3923-t6597)))+(t3.*t6719.*t7065)./1.0e+1;
et109 = -t3.*t8.*(t7610+t688.*(t6949+t6821.*(t1928-t4165)+t6741.*(t3626-t6712))+t3.*t4.*(t6813+t7165+t6760.*(t1928-t4165)));
et110 = t358+t523+t535+t696-t833+t933+t1007+t1660+t1865+t2152+t2221+t2343+t2648+t2899+t2988+t2990+t3007+t3039+t3262+t3330+t3543+t3587+t3809+t3872+t3892+t3922+t4044+t4095+t4203+t4316+t4374+t4646+t4675+t4844+t5148+t5955+t7369.*(t304+t372+t405+t418-t566+t740+t748-t782+t1309+t1505-t12.*t101.*(3.0./1.0e+1)-t12.*t106.*(3.0./1.0e+1))-t9.*t8132+t7363.*(t214./1.0e+1+t370+t401+t408+t460-t565+t735-t852+t1053+t1339+t1585-(t8.*t110)./1.0e+1)-t7370.*(t200.*(3.0./1.0e+1)+t208.*(6.0./5.0)-t303-t415-t747-t1313+t12.*t105.*(3.0./1.0e+1)+t9.*t748)+t7201.*(t191.*(2.0./5.0)+t297+t413+t463+t504-t766-t850-t868+t1046+t1300+(t12.*t84)./1.0e+1-(t48.*t128)./1.0e+1);
et111 = t2.*t3.*(t7607-t7613+t7942+t688.*(t6826+t6880-t7180-t7182-t7216+t6797.*(t1552-t4983))+t10.*t7505+t3.*t4.*(t6725+t6783+t6977+t7035-t7048+t7122))+t5.*t6.*t11.*(3.0./5.0e+1)-t3.*t8.*t8212-(t3.*t6719.*t6764)./1.0e+1-(t3.*t6722.*t7065)./1.0e+1;
et112 = (t7201.*(t296+t369+t397+t404-t562+t728+t738-t768+t1301+t1500-(t12.*t101)./1.0e+1-(t12.*t106)./1.0e+1))./2.0-(t7200.*(t304+t372+t405+t418-t566+t740+t748-t782+t1309+t1505-t12.*t101.*(3.0./1.0e+1)-t12.*t106.*(3.0./1.0e+1)))./2.0-(t7365.*(t191.*(6.0./5.0)+t305+t425+t478+t505-t781-t793-t861-t879+t1308+t12.*t84.*(3.0./1.0e+1)-t48.*t128.*(3.0./1.0e+1)))./2.0+(t9.*(-t7684+t7777+t688.*(t6834-t6843+t6863+t6870-t6959+t1664.*(t3626-t6712))))./2.0+(t1250.*t8118)./2.0-(t7368.*t7370)./2.0+(t7367.*t7372)./2.0;
et113 = t688.*(t7896+t9.*(t6800+t6805+t6935-t6960-t6966+t6570.*(t1552-t4983))+t2.*t3.*(t6946+t6948-t6987-t7075+t6.*t3709.*(t1552-t4983).*1.0675e-2+t6.*t3709.*(t3626-t6712))).*(-1.0./2.0)-(t7362.*(t200.*(3.0./1.0e+1)+t208.*(6.0./5.0)-t303-t415-t747-t1313+t12.*t105.*(3.0./1.0e+1)+t9.*t748))./2.0+(t7366.*(t191.*(2.0./5.0)+t297+t413+t463+t504-t766-t850-t868+t1046+t1300+(t12.*t84)./1.0e+1-(t48.*t128)./1.0e+1))./2.0+(t7363.*(t208.*(2.0./5.0)-t295-t402-t736+t772+t1274+(t12.*t105)./1.0e+1-(t12.*t200)./1.0e+1))./2.0;
et114 = (t3.*t4.*(t7682-t7770+t2.*t3.*(t6834-t6843+t6863+t6870-t6959+t1664.*(t3626-t6712))))./2.0-(t2.*t3.*t8123)./2.0+(t3.*t8.*t8120)./2.0-t3.*t4528.*t7062.*(3.0./2.0e+1)+(t3.*t4528.*t7065)./2.0e+1-t3.*t6719.*t7063.*(3.0./2.0e+1)+(t3.*t6719.*t7066)./2.0e+1;
et115 = dq1.*(t647+t678+t703+t828+t893+t916+t973+t1004+t1023+t1034+t1080+t1182+t1243+t1287+t1361+t1388+t1430+t1460+t1481+t1528+t1543+t1686+t1697-t1829+t1874+t1933+t2132+t2141+t2168+t2409+t2507+t2580+t2586+t2594+t2625+t2655+t2785+t2795+t2938+t2949+t3002+t3040+t3150+t3209+t3220+t3283+t3335+t3471+t3492+t3566+t3567+t3598+t3599+t3608+t3697+t3885+t3932+t3953+t4016+t4037+t4137+t4200+t4212+t4244+t4282+t4305+t4319+t4385+t4533+t4536+t4539+t4631+t4644+t4674+t4756+t4778+t4780+t4852+t4880+t4919+t4921+t4930+t5032+t5036+t5061+t5085+t5143+t5156+t5191+t5277+t5295+t5296+t5298+t5413+t5461+t5475+t5482+t5501+t5529+t5545+t5573+t5576+t5595+t5622+t5679+t5778+t5804+t5906+t5971+t5989+t6010+t6051+t6179+t6188+t6262+t6270+t6357+t6366+t6405+t6443+t6449+t6640+t8056+t8060+t8163+t8165+t12.*t600+t12.*t1446)-dq6.*t7595-dq2.*t8255-dq3.*(et110+et111)+dq4.*(et112+et113+et114);
et116 = dq5.*(t182+t253+t664+t1005+t1245+t1479+t2086+t2097+t2248+t2451+t2615+t2732+t2733+t2792+t3016+t3033+t3079+t3238+t3604+t3677+t3776+t3904+t4036+t4048+t4317+t4850+t5292+t7128-t7129+t7229+t7313+t7316+t7348+t7477+t7479+t7530+t7541+t7972+t7973+t7974+t7985+t8025+t8031+t8053+t8054+t8066+t8068+t8094+t8101+t8112+t8113+t8122+t8125+t8134+t8217+t8220);
et117 = t55.*1.91295e+1-t60.*8.829-t107.*8.829-t123.*1.91295e+1;
et118 = t2486.*(t140+t1806+t2069+t2551+t2603+t2862+t3235-t7545.*(t304+t372+t405+t418-t566+t740+t748-t782+t1309+t1505-t12.*t101.*(3.0./1.0e+1)-t12.*t106.*(3.0./1.0e+1))-t690.*(t7435+t1250.*(t6874+t7086+t3756.*(t3923-t6597))+t688.*(-t6862+t7059+t3710.*(t3626-t6712)))+t6914.*t7065+t7363.*t7543+t3755.*(t7610+t688.*(t6949+t6821.*(t1928-t4165)+t6741.*(t3626-t6712))+t3.*t4.*(t6813+t7165+t6760.*(t1928-t4165)))+t3709.*(t7522+t7605+t1250.*(t6947+t6849.*(t1552-t4983)+t6740.*(t3923-t6597))));
et119 = t2483.*(t10.*1.039659375+t56.*(3.0./4.0e+2)+t58.*(3.0./5.0e+1)+t61.*(1.17e+2./2.0e+2)+t113.*(3.0./2.5e+1)-t129.*(3.0./1.0e+2)-t261-t610+t839+t1720+t2280+t2439+t2474+t2568+t2739+t2767+t2806+t2825+t2888+t3071+t3254+t3363+t3394+t3529+t3702+t3714+t3777+t3918+t3993+t4331+t4343+t4410+t4550+t4582+t4604+t4661+t4823+t4940+t5306+t5433+t5.*t10.*(2.7e+1./1.0e+2)-t10.*t21.*2.98328125e-2+t5.*t58.*(9.0./1.0e+2)-t5.*t62.*(9.0./2.0e+2)-t12.*t58.*(3.0./5.0e+1)-t21.*t56.*(3.0./5.0e+1)+t12.*t114.*2.98328125e-2)-t6.*t690.*2.943+t12.*t690.*1.4715;
et120 = -t2487.*t7286-t2482.*t8130+dq5.*(et100+et101+et102)-t2485.*(t92+t186+t360+t1256+t1959+t2087+t2125+t2324+t2362+t2411+t2743+t2815+t2821+t3256+t3364+t4056+1.039659375)-dq2.*(et103+et104+et105)-dq1.*(et106+et107)-dq4.*(dq6.*t7396+dq5.*(t141+t143+t267+t1868+t2023+t2067+t2478+t2727+t2863+t2996+t3588+t3621+t3856+t4243))-t2484.*(et108+et109)+dq3.*(et115+et116)-dq6.*(t7400+t7599+t7902+t8051+dq5.*t7323+dq6.*(t2078+t2543+t2892+t13.*t346.*5.625e-3))-t12.*t690.*t1006.*5.518125e-1-t212.*t346.*t1253.*5.518125e-1+t6.*t216.*t346.*t690.*5.518125e-1;
et121 = t98.*(3.0./5.0e+1)+t605+t606+t639+t947+t1032-t1073+t1092-t1118+t1149+t1180+t1194-t1394+t1411+t1416+t1429+t1442+t1542+t1676-t1735+t1755+t1764+t1816+t1820+t1840+t2000+t2003+t2038+t2127+t2179+t2223+t2229-t2237+t2588+t2692-t2703+t2910+t2911+t2939+t3068+t3070+t3104+t3159+t3195+t3247+t3271-t3308+t3323+t3416+t3474+t3522+t3609+t3612+t3691+t3780+t3861+t3874+t3876+t3884+t3982+t4019+t4103+t4119+t4123+t4142+t4143+t4208+t4245+t4252+t4361+t4384+t4403+t4444+t4538+t4649+t4671+t4729+t4747+t4757+t4805+t4816+t4818+t4831+t4838+t4858+t4879+t4898+t4918+t5048+t5062+t5153+t5161+t5278+t5328+t5364+t5412+t5417+t5445+t5465+t5532+t5536+t5561+t5579+t5612+t5646+t5648+t5678+t5701+t5735+t5747+t5753+t5803+t5836+t5896+t5905+t5969+t5974+t5987+t6026+t6029+t6043+t6063+t6130+t6136+t6139+t6161+t6178+t6201+t6216+t6313+t6363+t6386+t6404+t6435+t6442+t6447+t6475+t6481+t6487+t6531+t6576+t6635+t6655+t6657+t7445+t7547+t7556+t7720+t7746+t7750+t7879+t7880+t8018+t8020+t8074+t8076+t8172+t8175-t6.*t54.*(3.0./2.0e+2);
et122 = t20.*t110.*(9.0./2.0e+2)-t10.*t892-t12.*t982+t22.*t3323+t7.*t13.*t126.*5.5078125e-3-t10.*t20.*t966+t86.*t99.*t1256+t19.*t21.*t22.*t54.*5.5078125e-3+t7.*t13.*t19.*t98.*5.5078125e-3+t7.*t13.*t56.*t203.*5.5078125e-3-t3.*t4.*t20.*t700+t19.*t28.*t54.*t1256+t20.*t62.*t97.*t1256;
et123 = t141+t143+t267+t312+t331+t684+t692+t834+t1025+t1039+t1086+t1196+t1376+t1392+t1496+t1526+t1541+t1681+t1868+t1997+t2014+t2023+t2067+t2383+t2478+t2629+t2727+t2863+t2928+t2996+t3101+t3149+t3207+t3386+t3411+t3470+t3520+t3565+t3588+t3621+t3658+t3680+t3720+t3856+t3909+t3950+t4132+t4211+t4218+t4243+t4309+t4370+t4379+t4614+t4770+t4797+t4961+t5087+t5120+t5166+t5190+t5203+t5242+t5331+t5345+t5419+t5424+t5467+t5497+t5588+t5617+t5705+t5757+t5893+t6141+t6196+t6258+t6356+t6424+t6523+t6638+t7299.*(t108.*(3.0./1.0e+1)-t210.*(3.0./1.0e+1)-t384+t432+t488+t1068)-t6906.*t7304-t2.*(-t7618-t7884+t7929+t3709.*(t6829-t6885-t7144-t7153+t6821.*(t193-t2663)+t6151.*(t3626-t6712))+t1252.*(t6813+t7165+t6760.*(t1928-t4165))+t1661.*(t6949+t6821.*(t1928-t4165)+t6741.*(t3626-t6712)));
et124 = -t8.*(t7625+t7634+t7924-t7926+t690.*(t6766+t6817+t7016-t7130+t6760.*(t189-t2612)+t6790.*(t1552-t4983))+t1252.*(-t6799+t7137+t6786.*(t1552-t4983)))-t8.*t7299.*(t7195+t7239-t7290-t7390)+t2.*t7304.*t7553+t8.*t7304.*t7551+t2.*t7299.*t7885;
et125 = dq6.*t7721+dq3.*t8257+dq4.*(t113.*(-3.0./4.0e+1)+t129.*(3.0./2.0e+2)+t337+t1172+t1406+t1473+t1711+t1878+t2171+t2238+t2397+t2422+t2661+t2843+t2953+t3006+t3215+t3224+t3227+t3328+t3443+t3578+t3629+t3668+t3899+t4202+t4249+t4287+t4333+t4429+t4594+t4615+t4655+t4786+t5059+t5146+t5302+t5629+t5966+t7397+t7407+t7408+t7425+t7447+t7449+t7465+t7467+t7655+t7660+t7695+t7696+t7714+t7715+t7954+t7958+t7993+t7998+t8037+t8082+t8084+t8160+t8204+t8209+t8221+t8222)+dq1.*(et121+et122)-dq2.*(et123+et124);
et126 = dq5.*(t6905.*(t108.*(3.0./1.0e+1)-t210.*(3.0./1.0e+1)-t384+t432+t488+t1068).*(-1.0./2.0)+(t690.*t7420)./2.0+(t2.*t8115)./2.0+(t3709.*t7600)./2.0+(t3755.*t7602)./2.0-(t6906.*t6914)./2.0+(t6911.*t7304)./2.0-(t6910.*t7307)./2.0+(t8.*(-t7749+t7861+t3709.*(t7250+t7263+t6821.*(t1552-t4983)+t6740.*(t3242-t6692))))./2.0+t2.*t6914.*t7545.*(3.0./2.0)+t8.*t6914.*t7543.*(3.0./2.0)-(t2.*t6914.*t7553)./2.0-(t8.*t6914.*t7551)./2.0-t2.*t7299.*t7453.*(3.0./2.0)+(t2.*t7299.*t7455)./2.0-t8.*t7299.*(t7131-t7306).*(3.0./2.0)+(t8.*t7299.*(t7141-t7309))./2.0);
et127 = t98.*(3.0./5.0e+1)+t605+t606+t639+t947+t1032-t1073+t1092-t1118+t1149+t1180+t1194-t1394+t1411+t1416+t1429+t1442+t1542+t1676-t1735+t1755+t1764+t1816+t1820+t1840+t2000+t2003+t2038+t2127+t2179+t2223+t2229-t2237+t2588+t2692-t2703+t2910+t2911+t2939+t3068+t3070+t3104+t3159+t3195+t3247+t3271-t3308+t3323+t3416+t3474+t3522+t3609+t3612+t3691+t3780+t3861+t3874+t3876+t3884+t3982+t4019+t4103+t4119+t4123+t4142+t4143+t4208+t4245+t4252+t4361+t4384+t4403+t4444+t4538+t4649+t4671+t4729+t4747+t4757+t4805+t4816+t4818+t4831+t4838+t4858+t4879+t4898+t4918+t5048+t5062+t5153+t5161+t5278+t5328+t5364+t5412+t5417+t5445+t5465+t5532+t5536+t5561+t5579+t5612+t5646+t5648+t5678+t5701+t5735+t5747+t5753+t5803+t5836+t5896+t5905+t5969+t5974+t5987+t6026+t6029+t6043+t6063+t6130+t6136+t6139+t6161+t6178+t6201+t6216+t6313+t6363+t6386+t6404+t6435+t6442+t6447+t6475+t6481+t6487+t6531+t6576+t6635+t6655+t6657+t7445+t7547+t7556+t7720+t7746+t7750+t7879+t7880+t8018+t8020+t8074+t8076+t8172+t8175-t6.*t54.*(3.0./2.0e+2);
et128 = t20.*t110.*(9.0./2.0e+2)-t10.*t892-t12.*t982+t22.*t3323+t7.*t13.*t126.*5.5078125e-3-t10.*t20.*t966+t86.*t99.*t1256+t19.*t21.*t22.*t54.*5.5078125e-3+t7.*t13.*t19.*t98.*5.5078125e-3+t7.*t13.*t56.*t203.*5.5078125e-3-t3.*t4.*t20.*t700+t19.*t28.*t54.*t1256+t20.*t62.*t97.*t1256;
et129 = t8244-dq5.*((t3755.*(t7097+t7109+t6741.*(t1387-t3956)+t6726.*(t1928-t4165)))./2.0-(t3709.*(t4014.*t6821-t4014.*t6845+(t97-t1942).*(t3242-t6692)-(t97-t1942).*(t3626-t6712)))./2.0+(t3709.*t7698)./2.0+(t7221.*t7543)./2.0-(t7223.*t7545)./2.0-(t7220.*t7551)./2.0+(t7222.*t7553)./2.0-(t7415.*t7453)./2.0+(t7414.*t7455)./2.0+(t7419.*(t7131-t7306))./2.0-(t7416.*(t7141-t7309))./2.0-(t3755.*(t4014.*t6859+t6824.*(t97-t1942)-t6849.*(t97-t1942)+t4014.*(t3923-t6597)))./2.0)-dq6.*t7999+dq4.*t8253-dq2.*(et127+et128);
et130 = dq3.*(t202.*(3.0./5.0e+1)-t250-t260+t596+t638-t758+t889+t906+t1033+t1097+t1193+t1298+t1378+t1525+t1579+t1594+t1678+t1754+t1763+t1772+t1785+t1839+t2002+t2138+t2866+t2960+t3037+t3129+t3152+t3413+t3454+t3472+t3480+t3568+t3655+t3764+t3814+t3829+t3860+t3901+t4121+t4168+t4276+t4454+t4551+t4712+t4733+t4775+t4804+t4860+t4917+t5010+t5193+t5244+t5326+t5411+t5416+t5426+t5513+t5749+t5897+t5930+t5964+t6025+t6042+t6115+t6120+t6138+t6150+t6160+t6352+t6358+t6403+t6434+t6441+t7424+t7550+t7562+t7666+t7758+t7759+t7852+t7856+t8006+t8013+t8077+t8080+t8176+t8178+t51.*t441+t6.*t9.*t20.*(3.0./2.0e+2)+t9.*t12.*t20.*(3.0./1.0e+2));
et131 = t7453.*(t191.*(6.0./5.0)+t305+t425+t478+t505-t781-t793-t861-t879+t1308+t12.*t84.*(3.0./1.0e+1)-t48.*t128.*(3.0./1.0e+1)).*(-1.0./2.0)-(t3709.*t8104)./2.0+(t7213.*t7545)./2.0-(t7212.*t7553)./2.0-(t7225.*t7543)./2.0+(t7224.*t7551)./2.0+(t690.*(t7606-t7702+t3.*t8.*(t7060-t7088+t7104+t3710.*(t3923-t6597))))./2.0+(t7372.*(t7131-t7306))./2.0-(t7370.*(t7141-t7309))./2.0+(t7455.*(t191.*(2.0./5.0)+t297+t413+t463+t504-t766-t850-t868+t1046+t1300+(t12.*t84)./1.0e+1-(t48.*t128)./1.0e+1))./2.0;
et132 = (t9.*(-t7639+t7723+t3755.*(t7060-t7088+t7104+t3710.*(t3923-t6597))))./2.0-(t3755.*(-t7813+t9.*(t7138-t7166+t7176+t6757.*(t1928-t4165))+t3.*t8.*(t7257+t7267+t6824.*(t1928-t4165)+t6741.*(t3923-t6597))))./2.0+(t3.*t4219.*(t108.*(3.0./1.0e+1)-t210.*(3.0./1.0e+1)-t384+t432+t488+t1068))./2.0e+1+(t3.*t8.*t8115)./2.0+t3.*t4219.*t6914.*(3.0./2.0e+1)+t3.*t6719.*t6910.*(3.0./2.0e+1)-(t3.*t6719.*t6911)./2.0e+1-(t2.*t3.*(-t7749+t7861+t3709.*(t7250+t7263+t6821.*(t1552-t4983)+t6740.*(t3242-t6692))))./2.0;
et133 = t183+t186+t494+t527+t531+t913+t1041+t1383+t2457+t2651+t2848+t2900+t2992+t3091+t3239+t3395+t3752+t4013+t4029+t4162+t4377+t4435+t4595+t5208+t5293+t5526+t5956+t7369.*t7553-t7370.*t7862-t7551.*(t214./1.0e+1+t370+t401+t408+t460-t565+t735-t852+t1053+t1339+t1585-(t8.*t110)./1.0e+1)+t9.*(t7443-t7667+t3709.*(t6784+t6806-t6978+t6981+t7021+t7024)+t3755.*(t6792+t6809-t6979+t6982+t7022+t7025)+t2027.*(t6874+t7086+t3756.*(t3923-t6597))+t1662.*(-t6862+t7059+t3710.*(t3626-t6712)))+t7870.*(t191.*(2.0./5.0)+t297+t413+t463+t504-t766-t850-t868+t1046+t1300+(t12.*t84)./1.0e+1-(t48.*t128)./1.0e+1);
et134 = -t2.*t3.*(t7626+t7825+t7946+t3709.*(t6826+t6880-t7180-t7182-t7216+t6797.*(t1552-t4983))+t2027.*(t6947+t6849.*(t1552-t4983)+t6740.*(t3923-t6597))+t4.*t49.*(-t6799+t7137+t6786.*(t1552-t4983)))-(t3.*t6722.*(t108.*(3.0./1.0e+1)-t210.*(3.0./1.0e+1)-t384+t432+t488+t1068))./1.0e+1+t3.*t8.*t8224+(t3.*t6719.*t6776)./1.0e+1;
et135 = dq5.*(et131+et132)+dq6.*t7434+dq2.*t8257+dq4.*(t182+t253+t664+t1005+t1245+t1479+t2086+t2097+t2248+t2451+t2615+t2732+t2733+t2792+t3016+t3033+t3079+t3238+t3604+t3677+t3776+t3904+t4036+t4048+t4317+t4850+t5292-t7128+t7129+t7230-t7311+t7315+t7346-t7473+t7480+t7529+t7703+t7713+t7978+t7981+t7984+t7988+t8036+t8085+t8088+t8105+t8137+t8141+t8205+t8211+t8228+t8230+(t7213.*(t296+t369+t397+t404-t562+t728+t738-t768+t1301+t1500-(t12.*t101)./1.0e+1-(t12.*t106)./1.0e+1))./2.0+(t1250.*(-t7813+t9.*(t7138-t7166+t7176+t6757.*(t1928-t4165))+t3.*t8.*(t7257+t7267+t6824.*(t1928-t4165)+t6741.*(t3923-t6597))))./2.0+(t3.*t4.*(t7606-t7702+t3.*t8.*(t7060-t7088+t7104+t3710.*(t3923-t6597))))./2.0);
et136 = -dq1.*(t202.*(3.0./5.0e+1)-t250-t260+t596+t638-t758+t889+t906+t1033+t1097+t1193+t1298+t1378+t1525+t1579+t1594+t1678+t1754+t1763+t1772+t1785+t1839+t2002+t2138+t2866+t2960+t3037+t3129+t3152+t3413+t3454+t3472+t3480+t3568+t3655+t3764+t3814+t3829+t3860+t3901+t4121+t4168+t4276+t4454+t4551+t4712+t4733+t4775+t4804+t4860+t4917+t5010+t5193+t5244+t5326+t5411+t5416+t5426+t5513+t5749+t5897+t5930+t5964+t6025+t6042+t6115+t6120+t6138+t6150+t6160+t6352+t6358+t6403+t6434+t6441+t7424+t7550+t7562+t7666+t7758+t7759+t7852+t7856+t8006+t8013+t8077+t8080+t8176+t8178+t51.*t441+t6.*t9.*t20.*(3.0./2.0e+2)+t9.*t12.*t20.*(3.0./1.0e+2))+dq3.*(et133+et134);
et137 = (t7455.*(t296+t369+t397+t404-t562+t728+t738-t768+t1301+t1500-(t12.*t101)./1.0e+1-(t12.*t106)./1.0e+1))./2.0-(t7453.*(t304+t372+t405+t418-t566+t740+t748-t782+t1309+t1505-t12.*t101.*(3.0./1.0e+1)-t12.*t106.*(3.0./1.0e+1)))./2.0+(t6770.*(t108.*(3.0./1.0e+1)-t210.*(3.0./1.0e+1)-t384+t432+t488+t1068))./2.0-(t690.*t8093)./2.0-(t1250.*t8115)./2.0+(t3709.*t8108)./2.0+(t6771.*t6914)./2.0-(t6911.*t7062)./2.0+(t6910.*t7065)./2.0-(t7020.*t7545)./2.0+(t7027.*t7543)./2.0+(t7019.*t7553)./2.0-(t7026.*t7551)./2.0+(t7363.*(t7131-t7306))./2.0-(t7362.*(t7141-t7309))./2.0;
et138 = t688.*(-t7749+t7861+t3709.*(t7250+t7263+t6821.*(t1552-t4983)+t6740.*(t3242-t6692))).*(-1.0./2.0)+(t3755.*(t7838+t1250.*(t7257+t7267+t6824.*(t1928-t4165)+t6741.*(t3923-t6597))+t3.*t4.*(t7138-t7166+t7176+t6757.*(t1928-t4165))))./2.0-(t3.*t4.*(-t7639+t7723+t3755.*(t7060-t7088+t7104+t3710.*(t3923-t6597))))./2.0;
et139 = dq3.*(t182+t253+t664+t1005+t1245+t1479+t2086+t2097+t2248+t2451+t2615+t2732+t2733+t2792+t3016+t3033+t3079+t3238+t3604+t3677+t3776+t3904+t4036+t4048+t4317+t4850+t5292+t7230+t7313+t7315+t7346+t7477+t7479+t7530+t7541+t7703+t7713+t7978+t7981+t7984+t7988+t8036+t8085+t8088+t8094+t8112+t8113+t8137+t8141+t8205+t8211+t8228+t8230)-dq6.*t7361-dq1.*t8253+dq5.*(et137+et138);
et140 = -dq4.*(t141+t143+t267+t1868+t2023+t2067+t2478+t2727+t2863+t2996+t3588+t3621+t3856+t4243+t7063.*(t108.*(3.0./1.0e+1)-t210.*(3.0./1.0e+1)-t384+t432+t488+t1068)+t1250.*t8199-t6771.*t7062+t7365.*t7553+t7367.*t7551-t7362.*t7866-(t7249-t7282-t7389+t3755.*(t166+t298+t2276-t2308).*3.0).*(t296+t369+t397+t404-t562+t728+t738-t768+t1301+t1500-(t12.*t101)./1.0e+1-(t12.*t106)./1.0e+1)-t688.*(t7559+t7642+t7644-t7923+t3709.*(t6946+t6948-t6987-t7075+t6.*t3709.*(t1552-t4983).*1.0675e-2+t6.*t3709.*(t3626-t6712))+t690.*(t6800+t6805+t6935-t6960-t6966+t6570.*(t1552-t4983)))+t3.*t4.*t8140);
et141 = dq2.*(t252+t261+t530+t557+t610+t700+t904+t912+t950+t1075+t1172+t1878+t2171+t2238+t2397+t2422+t2491+t2610+t2661+t2843+t2905+t2953+t3006+t3215+t3224+t3227+t3328+t3443+t3578+t3629+t3668+t3899+t4202+t4249+t4287+t4333+t4429+t4594+t4615+t4655+t4786+t5059+t5146+t5302+t5629+t5966-t7393+t7397+t7407+t7695+t7696+t7714+t7715+t7954+t7958+t7993+t7998+t8037+t8082+t8084+t8160+t8204+t8209+t8221+t8222);
et142 = t97.*2.943-t108.*1.4715-t1930.*1.4715-t1942.*2.943-dq2.*(et125+et126)-dq6.*(t6665+t7378+t7441+t7722+t8002+dq6.*t7.*t3194.*5.859375e-5)+t2486.*(t29.*5.5078125e-3-t2743+t29.*t1323-9.7159375e-2)-dq6.*t6665+dq1.*(et129+et130)+t1006.*t4014.*5.518125e-1;
et143 = t2485.*(t140+t1806+t2069+t2551+t2603+t2862+t3235-t7553.*(t296+t369+t397+t404-t562+t728+t738-t768+t1301+t1500-(t12.*t101)./1.0e+1-(t12.*t106)./1.0e+1)-t7062.*(t108.*(3.0./1.0e+1)-t210.*(3.0./1.0e+1)-t384+t432+t488+t1068)+t688.*t8073+t1250.*t8072+t7362.*t7551+t3.*t4.*(-t7450+t3755.*(t6874+t7086+t3756.*(t3923-t6597))+t3709.*(-t6862+t7059+t3710.*(t3626-t6712))));
et144 = t2484.*(t245+t263+t667+t1484+t1926+t1949+t2403+t2477+t2811+t3255+t3379+t3444+t3671+t3888+t3919+t7370.*t7551-t9.*(-t7450+t3755.*(t6874+t7086+t3756.*(t3923-t6597))+t3709.*(-t6862+t7059+t3710.*(t3626-t6712)))-t7553.*(t191.*(2.0./5.0)+t297+t413+t463+t504-t766-t850-t868+t1046+t1300+(t12.*t84)./1.0e+1-(t48.*t128)./1.0e+1)-(t3.*t6719.*(t108.*(3.0./1.0e+1)-t210.*(3.0./1.0e+1)-t384+t432+t488+t1068))./1.0e+1+t2.*t3.*t8073-t3.*t8.*t8072)-dq3.*(et135+et136)-dq4.*(et139+et140+et141);
et145 = -t2483.*(t244+t341+t496+t609+t1157+t1163+t1860+t2111+t2212+t2400+t2440+t2964+t3043+t3098+t3099+t3442+t3679+t3703+t3852+t3887+t3906+t3994+t4195+t4292+t4507+t4603+t4868+t5066-t7304.*(t108.*(3.0./1.0e+1)-t210.*(3.0./1.0e+1)-t384+t432+t488+t1068)+t2.*t8072+t8.*t8073+t2.*t7299.*t7553+t8.*t7299.*t7551)-t2482.*(t387+t511+t637+t890+t945+t1090+t1189+t1334+t1787+t1883+t2148+t2231+t2254+t2259+t2565+t2878+t2943+t3004+t3050+t3348+t3353+t3533+t3767+t3916+t4092+t4311+t4313+t4341+t4428+t4493+t4597+t4641+t4658+t4670+t4710+t4754+t4807+t5030+t5095+t5384+t5436+t5547+t5637+t7427-t3755.*t7486+t7414.*t7553-t7416.*t7551-t3709.*(-t6862+t6821.*(t97-t1942)+t4014.*(t3626-t6712)))+t13.*t2487.*t3194.*5.859375e-5-t216.*t346.*(t97-t1942).*5.518125e-1;
et146 = dq1.*(t8236+dq5.*t7999+dq4.*t8046+dq2.*t8202-dq3.*(t1609+t1619+t2103+t2157+t2348+t2401+t2527+t2536+t2574+t2672+t2764+t2772+t2832+t3147+t3366+t3438+t3467+t3481+t3488+t3663+t3807+t3831+t3970+t4084+t4183+t4233+t4391+t4419+t4574+t4633+t4817+t5039+t5094+t5136+t5187+t5215+t5223+t5389+t5449+t5498+t5510+t5609+t5676+t5722+t5729+t5910+t6055+t6091+t6340+t11.*t3073+t9.*t20.*t2222+t11.*t112.*t2324+t9.*t13.*t3214-t7.*t9.*t13.*t20.*5.5078125e-3+t9.*t20.*t21.*t2222-t7.*t9.*t13.*t20.*t21.*5.5078125e-3))+dq4.*(t7400+t7599+t7902+t8051-dq5.*t7361)-t2485.*t7286-t2484.*t7403+t2483.*t7725+t2482.*t7966+dq5.*(t6665+t7378+t7441+t7722+t8002)-t2487.*(t1323+5.9765625e-3)-dq3.*(t7802+t8052+t8117-dq5.*t7434-dq4.*t7595);
et147 = dq2.*(t8097+t8206+dq5.*t7721-dq3.*t8050+dq4.*(t1613+t1620-t2161+t2185+t2395+t2405+t2578+t2679+t3436-t3442+t3882-t4007+t4399+t4496+t21.*t1804+t21.*t2598+t21.*t2601-t22.*t63.*t113.*1.376953125e-3-t7.*t10.*t346.*(9.0./3.2e+2)-t12.*t13.*t58.*t63.*2.75390625e-3-t12.*t13.*t58.*t346.*5.625e-3-t13.*t21.*t56.*t346.*5.625e-3))+t216.*t346.*t690.*5.518125e-1-t212.*t346.*t4014.*5.518125e-1+t13.*t2486.*t3194.*5.859375e-5;
tau = [et36+et37+et38;et64+et65+et66+et67+et68;et90+et91+et92+et93+et94+et95+et96;et117+et118+et119+et120;et142+et143+et144+et145;et146+et147];
end
